simulink model "day06p2"  (R2026a)
settings: Solver=VariableStepAuto  StopTime=inf
InitFcn:
  | input = [9 0 0 0 1 1 0 7 1 0 0 0 4 5 0 3 6 0 2 3 8 4 0 9 9 4 0 6 5 7 0 0 7 7 2 0 8 2 6 0 4 5 2 5 0 1 3 9 1 0 0 9 3 0 1 6 0 0 0 7 0 3 3 0 1 6 9 0 8 3 1 1 0 8 8 0 7 1 0 1 0 0 5 8 0 0 8 0 5 4 0 8 3 0 0 0 7 0 5 4 9 0 0 9 0 6 8 4 0 2 7 0 7 9 1 0 1 2 8 0 2 1 5 0 0 9 8 1 0 4 6 9 0 7 2 0 4 6 0 1 3 9 0 3 0 0 0 9 4 0 0 0 5 3 0 7 6 6 4 0 3 4 0 4 5 0 9 3 0 9 9 0 0 0 9 0 1 5 2 0 5 1 0 8 4 0 1 3 0 4 4 4 8 0 0 0 3 9 0 8 3 0 0 8 2 6 0 8 4 0 4 1 7 0 1 2 6 2 0 4 2 4 5 0 5 2 3 0 0 6 0 3 9 9 0 0 8 3 0 0 2 0 2 8 5 0 7 9 0 0 3 8 0 0 0 9 1 0 6 0 0 2 7 8 0 5 0 0 7 4 0 5 0 0 0 0 2 0 7 8 5 6 0 4 3 0 1 5 6 0 9 0 0 0 9 8 0 9 5 4 4 0 3 4 5 0 1 9 8 0 6 6 0 1 0 0 5 8 0 3 9 0 3 0 0 0 0 9 0 4 8 0 3 2 1 0 6 0 0 6 6 5 7 0 8 0 0 6 7 5 0 4 2 6 4 0 5 0 0 0 2 4 2 1 0 0 3 7 0 2 6 8 0 6 0 0 0 7 3 9 0 5 2 8 0 9 5 0 0 3 4 4 0 4 3 9 0 9 1 0 9 7 4 0 0 4 6 0 0 3 5 0 9 9 0 8 9 0 1 7 2 0 7 4 0 6 1 2 0 0 0 8 0 0 8 3 0 9 6 3 0 0 9 0 0 1 8 0 4 9 0 6 6 0 7 2 9 0 1 5 9 0 2 3 6 0 7 2 0 4 2 7 0 8 1 0 5 8 1 0 6 4 0 7 7 0 2 7 7 0 7 7 0 0 0 8 0 3 6 0 4 6 0 6 4 1 0 0 8 0 4 0 0 5 0 0 9 2 4 4 0 0 0 8 0 4 3 0 2 5 0 3 0 0 0 0 7 7 6 4 0 8 3 0 0 1 2 0 7 6 8 0 9 2 0 9 8 0 5 4 0 7 1 0 9 0 0 0 9 8 0 5 7 0 2 7 0 0 4 1 8 0 0 0 1 0 0 0 0 4 0 2 2 0 6 9 2 0 8 9 0 1 0 0 2 1 3 3 0 0 6 3 0 0 0 4 0 2 9 8 6 0 7 8 0 0 0 6 6 0 3 1 4 0 9 1 2 0 0 5 0 9 8 0 0 3 0 7 6 2 0 1 1 7 0 1 0 0 6 4 5 0 6 2 0 2 8 0 3 3 0 9 0 0 0 0 9 3 2 0 1 1 0 1 8 0 7 0 0 0 7 2 0 9 7 9 0 6 9 3 0 2 2 7 4 0 0 9 0 7 4 8 8 0 8 5 6 0 4 7 2 1 0 5 9 7 1 0 5 9 1 0 0 1 0 7 2 0 2 0 0 0 1 3 1 0 0 0 0 7 0 4 4 0 0 1 3 0 2 6 0 6 9 0 8 7 0 5 0 0 5 6 6 7 0 7 8 4 0 0 0 0 8 0 0 8 1 0 0 2 7 0 2 8 0 0 0 9 3 0 8 8 0 0 0 7 0 6 2 0 3 9 9 0 8 5 1 0 0 9 6 3 0 5 2 0 7 9 2 0 0 2 1 0 1 0 0 0 1 7 0 0 6 7 0 1 9 3 0 1 8 9 8 0 9 6 0 5 9 0 0 4 3 0 0 0 2 4 0 8 5 0 0 1 5 0 0 4 0 8 3 2 0 3 2 0 0 0 2 0 4 3 9 0 0 0 2 5 0 0 2 0 0 7 0 9 7 0 0 0 3 0 0 4 0 8 1 9 0 7 0 0 0 6 3 0 8 4 3 1 0 0 0 7 8 0 0 0 2 0 1 2 3 9 0 9 6 2 0 4 3 0 1 3 0 0 0 0 0 9 1 0 2 1 0 8 5 9 3 0 6 3 0 2 0 0 0 3 0 0 5 0 1 4 0 0 2 6 7 0 7 9 1 1 0 1 7 2 0 3 6 7 9 0 0 0 7 0 4 3 0 9 9 4 0 4 0 0 0 0 3 4 0 2 7 4 0 3 5 0 6 0 0 0 3 3 8 8 0 0 0 6 0 0 2 6 0 1 9 9 0 8 1 0 9 9 0 0 4 0 0 8 6 0 8 7 0 1 6 2 0 0 4 2 0 9 0 0 9 8 0 0 9 2 0 5 3 1 0 7 8 6 0 5 2 0 0 1 9 0 8 9 0 1 3 0 0 0 8 1 6 7 0 0 1 0 7 4 0 4 7 5 0 6 1 0 0 0 7 0 3 6 7 2 0 8 6 0 5 5 0 9 6 0 1 2 0 7 9 7 3 0 1 5 9 0 0 1 0 8 9 0 6 3 9 0 1 9 6 0 3 9 0 6 8 0 6 8 4 0 0 2 5 0 3 0 0 0 7 4 0 8 0 0 9 0 0 0 7 0 0 2 3 7 0 3 7 0 3 2 0 1 0 0 0 0 4 9 1 0 0 9 6 0 2 7 2 0 0 8 0 2 7 7 0 1 3 4 0 0 3 0 0 7 0 6 2 4 0 3 4 9 7 0 2 2 2 0 4 4 0 7 0 0 2 0 0 0 0 0 4 4 0 5 9 0 5 6 4 6 0 2 2 7 0 3 6 6 0 3 4 9 0 1 0 0 9 8 0 8 0 0 0 5 0 0 0 3 6 0 4 1 0 5 4 0 0 9 8 0 0 3 0 1 8 7 0 4 4 6 0 0 5 0 4 2 2 0 4 6 0 0 3 5 0 6 8 8 0 1 0 0 0 4 6 2 0 0 0 3 0 8 5 4 0 3 1 0 9 2 5 8 0 4 6 0 0 0 0 3 5 0 3 3 0 0 5 7 0 5 3 6 0 2 9 9 0 9 3 0 8 5 4 6 0 7 8 6 0 8 5 2 1 0 8 7 0 4 7 0 3 1 0 0 0 2 0 0 4 0 7 2 0 0 1 0 0 3 6 0 5 3 6 0 2 0 0 6 5 9 0 8 6 0 0 0 4 1 1 0 6 6 0 6 0 0 6 0 0 7 9 7 7 0 0 5 0 4 1 0 9 5 5 0 8 0 0 3 2 0 0 9 9 5 0 5 7 0 0 9 5 0 2 8 5 4 0 8 2 0 0 9 6 4 0 2 1 3 0 1 1 0 4 4 0 8 1 6 4 0 6 1 0 0 0 9 3 3 0 6 7 0 5 1 0 1 2 7 0 1 0 0 0 0 0 4 0 5 0 0 4 2 0 5 7 0 3 3 8 3 0 0 9 0 0 0 7 0 7 5 4 0 9 1 6 0 3 7 0 1 8 8 0 2 8 0 0 6 8 1 4 0 9 0 0 5 5 0 0 0 5 7 0 9 6 0 0 2 4 0 1 0 0 0 0 6 0 2 3 3 0 5 6 0 3 7 0 4 9 0 7 8 0 6 4 0 5 3 7 0 2 7 7 0 0 4 0 0 0 4 8 0 2 5 3 7 0 0 5 4 0 0 0 3 0 2 2 1 0 1 6 0 3 4 0 8 6 4 0 4 1 0 0 0 0 6 0 8 6 1 7 0 8 1 6 0 1 1 0 0 9 0 0 3 4 0 7 0 0 4 3 1 3 0 4 5 0 4 6 7 0 1 5 0 8 4 8 8 0 0 0 2 0 7 9 0 2 2 6 0 0 7 0 6 0 0 0 6 6 0 0 7 5 9 0 0 0 8 0 2 5 7 0 1 6 4 0 7 9 0 2 8 8 0 0 1 3 6 0 0 8 1 0 4 9 7 7 0 4 8 2 0 0 8 0 0 7 0 7 9 0 1 4 2 0 1 8 0 7 6 0 4 1 0 4 4 5 7 0 6 3 0 5 5 1 5 0 3 4 0 7 9 0 0 0 1 0 3 5 0 0 5 8 3 0 0 4 1 0 1 7 9 8 0 5 8 3 0 6 7 0 5 8 1 0 1 5 0 0 7 0 5 4 0 5 1 0 9 6 0 0 5 2 0 2 2 5 0 4 9 5 0 0 0 8 0 6 7 0 4 0 0 0 8 1 9 9 0 8 4 1 0 9 2 5 4 0 2 7 1 0 9 4 2 0 3 8 7 0 4 5 2 0 8 2 4 0 5 3 8 0 1 4 0 9 6 9 0 4 2 0 4 6 5 0 2 2 0 2 1 0 8 3 8 9 0 5 4 8 0 0 8 8 0 2 5 0 8 7 8 0 5 7 9 0 2 7 3 6 0 9 0 0 0 0 1 0 4 2 0 5 3 3 0 7 8 7 0 8 5 8 0 4 0 0 0 5 3 0 3 5 2 0 0 6 0 5 2 0 6 7 9 0 0 2 0 0 0 7 4 3 0 1 3 6 0 5 3 0 2 6 0 9 6 0 7 5 3 0 7 3 0 7 2 0 1 9 0 9 1 0 2 5 7 0 1 9 0 2 3 4 0 4 6 0 8 1 0 0 2 7 1 3 0 5 8 5 0 4 7 7 0 3 2 4 0 0 4 8 0 1 7 5 7 0 0 0 5 1 0 0 0 0 5 0 1 5 0 8 0 0 3 1 4 0 3 2 0 0 8 4 0 3 0 0 4 5 4 0 6 8 3 0 0 7 0 6 5 0 6 2 0 4 1 0 2 6 8 7 0 5 1 4 0 4 2 3 0 6 2 0 3 4 4 0 5 0 0 8 1 0 5 1 0 7 9 7 0 0 3 3 7 0 7 6 6 7 0 7 2 2 0 7 2 7 0 0 1 0 7 6 0 5 9 2 0 7 7 0 1 3 0 3 7 6 0 0 4 8 0 9 4 0 4 8 0 3 0 0 9 0 0 0 0 0 7 0 8 8 0 3 6 0 8 1 3 0 3 7 3 0 6 6 5 0 9 4 7 8 0 9 8 4 0 2 3 0 0 0 0 4 0 0 0 4 0 2 5 8 5 0 5 3 0 8 8 9 0 0 3 0 6 9 0 0 0 5 6 0 6 2 0 1 3 0 1 8 4 0 4 3 0 8 0 0 0 0 0 0 9 0 0 7 0 4 5 8 0 5 0 0 0 2 8 4 0 6 2 0 6 9 3 1 0 4 8 0 7 0 0 9 6 3 0 1 0 0 0 3 0 0 3 6 0 0 7 1 0 1 9 9 3 0 7 9 5 0 7 0 0 0 9 4 5 0 0 8 8 0 0 0 0 8 0 1 5 1 9 0 6 2 4 0 0 3 8 0 7 6 2 0 1 4 0 0 0 2 0 1 4 3 0 6 2 0 0 7 4 0 1 8 0 0 0 7 0 8 2 0 3 6 0 1 9 2 0 8 8 5 0 4 8 1 0 5 7 8 0 7 8 7 0 2 4 1 2 0 2 9 0 0 9 4 0 7 2 7 0 9 1 9 0 2 6 0 0 0 1 3 0 8 5 4 0 7 5 4 0 5 2 2 0 2 3 0 0 4 5 0 9 0 0 0 2 9 8 0 1 3 0 0 0 0 8 1 0 5 6 0 4 9 3 0 6 7 0 6 3 6 0 1 3 1 0 1 6 5 0 0 2 3 0 0 5 0 9 1 2 0 2 4 0 2 2 3 0 6 5 5 0 0 5 0 0 6 8 0 0 3 0 4 9 5 0 1 9 4 0 0 9 4 5 0 3 7 1 0 8 0 0 3 5 0 0 0 1 3 0 0 7 7 0 1 9 0 6 8 2 7 0 6 1 4 0 6 4 6 0 8 1 6 0 0 1 0 0 0 0 9 0 4 6 6 0 2 5 7 0 9 1 0 0 6 2 0 0 3 7 0 0 5 0 9 7 7 0 2 4 7 4 0 9 8 0 8 4 2 0 0 8 4 0 8 1 1 0 0 9 0 1 2 0 8 1 5 0 0 2 0 8 1 0 7 1 0 0 4 2 0 0 3 1 0 6 9 2 0 5 1 7 0 8 7 2 0 8 8 2 0 0 0 0 7 0 6 4 0 1 7 1 4 0 2 7 0 6 9 0 0 8 0 4 1 0 8 2 8 3 0 1 5 0 1 4 0 6 2 0 8 5 0 0 7 3 0 0 0 9 1 0 7 7 0 7 9 0 2 7 5 0 0 6 4 0 0 8 7 5 7 0 2 4 7 0 6 9 1 1 0 5 4 0 5 4 4 0 6 7 0 0 6 3 0 4 6 1 4 0 0 0 0 2 0 2 5 2 0 2 4 6 0 3 1 5 0 8 0 0 0 0 5 1 0 7 9 4 0 3 5 0 5 1 0 2 8 0 3 6 6 0 5 4 0 6 9 0 4 1 0 3 4 9 0 5 7 0 9 9 3 0 9 0 0 7 4 0 8 1 0 4 2 0 4 4 0 4 0 0 5 6 0 0 0 1 0 8 8 0 9 1 0 0 5 8 3 0 0 0 8 0 6 6 0 9 7 9 0 9 1 3 0 0 2 0 6 2 7 0 4 2 0 9 9 9 6 0 9 4 9 0 0 0 9 0 7 1 0 0 0 3 1 0 0 1 3 0 2 7 0 9 6 6 3 0 9 3 6 0 3 5 0 0 9 5 3 0 5 4 0 3 3 0 0 5 2 0 0 0 3 8 0 7 7 0 3 7 7 0 8 0 0 9 1 0 0 1 0 7 5 0 8 9 4 0 9 7 7 4 0 0 3 2 0 0 9 3 0 5 1 0 9 4 0 9 4 3 0 7 5 6 0 3 0 0 8 4 0 0 0 9 0 2 1 0 0 0 9 8 0 9 8 2 0 9 3 9 0 5 1 0 6 7 0 5 4 0 4 3 0 0 1 3 9 0 5 3 0 0 7 3 4 0 0 7 0 4 9 0 2 9 3 5 0 0 7 0 0 8 0 0 0 6 8 0 0 7 8 0 6 7 0 0 1 0 3 0 0 0 0 9 0 8 0 0 6 6 5 0 8 6 0 7 7 4 5 0 4 4 5 7 0 2 4 0 3 9 0 3 9 1 0 2 7 0 8 8 0 0 5 0 0 0 5 3 0 3 1 0 4 4 0 0 7 0 9 6 0 0 7 5 0 3 3 4 1 0 9 2 9 0 0 0 5 7 0 4 5 0 2 5 0 7 2 0 0 0 0 6 0 9 9 0 0 6 5 0 9 9 0 3 5 9 0 0 7 5 0 8 2 7 0 1 5 0 3 5 1 0 0 6 9 0 4 1 0 3 0 0 0 8 0 6 0 0 8 6 2 0 4 6 0 9 8 3 8 0 2 8 0 4 4 0 4 7 0 2 6 3 0 2 8 0 4 0 0 0 0 7 8 0 0 4 0 5 6 0 0 2 2 3 0 0 1 0 0 8 0 0 8 1 0 6 1 0 3 0 0 4 1 6 0 4 1 9 0 8 4 7 6 0 2 1 0 7 1 4 0 1 5 8 0 8 2 0 0 8 0 0 1 0 0 0 7 0 0 2 2 8 0 9 1 1 0 4 6 6 3 0 6 6 1 0 1 5 0 1 2 6 1 0 0 0 6 3 0 0 0 8 0 3 4 9 0 2 6 0 9 5 0 9 3 0 9 1 9 4 0 5 9 0 2 2 4 0 1 6 8 9 0 3 3 0 7 8 0 6 3 0 3 6 1 0 4 1 4 0 0 2 3 0 8 6 0 9 0 0 0 0 4 0 8 6 4 0 7 3 2 0 4 9 0 1 3 3 0 4 4 9 0 0 4 0 0 7 2 0 0 3 0 9 7 0 0 0 8 3 0 0 9 0 5 4 0 0 6 3 0 6 0 0 0 0 7 0 8 1 7 1 0 9 8 6 4 0 8 8 4 0 4 4 8 0 8 7 1 0 8 6 5 0 9 4 0 0 0 7 2 0 5 7 6 0 9 9 0 5 2 0 0 3 0 0 5 8 0 0 0 7 2 0 8 9 4 0 1 5 0 6 6 0 7 2 0 5 5 2 7 0 6 0 0 0 9 4 0 0 1 0 0 5 5 9 0 0 0 5 0 1 7 5 0 8 5 0 3 9 0 0 0 3 0 2 7 0 0 5 0 7 0 0 9 2 0 0 0 0 8 0 7 2 8 0 0 0 3 0 8 0 0 0 4 7 3 0 2 7 4 0 0 3 4 0 7 2 0 5 6 9 9 0 3 9 0 9 2 0 5 4 4 7 0;
  |     1 5 0 0 9 5 0 6 8 6 0 0 6 3 0 6 5 0 2 7 9 7 0 7 8 5 0 7 7 2 8 0 2 4 4 0 7 7 6 0 1 8 7 9 0 2 5 7 0 0 0 9 7 0 7 1 0 0 8 7 0 2 7 0 4 5 0 0 3 3 8 3 0 2 5 0 8 6 0 1 6 0 2 5 0 6 6 0 1 5 0 1 8 0 5 8 4 0 5 7 1 0 3 5 0 9 3 2 0 4 8 0 9 6 7 0 6 2 6 0 9 3 9 0 0 8 4 2 0 7 9 5 0 1 6 0 1 3 0 4 5 4 0 5 3 0 4 3 3 0 0 2 6 3 0 8 4 5 8 0 9 2 0 6 1 0 4 1 0 1 4 5 0 0 5 0 6 4 9 0 7 9 0 8 4 0 2 0 0 3 5 1 5 0 0 7 6 4 0 6 9 0 0 8 7 6 0 4 8 0 6 5 3 0 8 8 9 9 0 4 3 1 3 0 9 3 0 0 3 1 0 8 2 8 0 0 9 1 0 9 3 0 4 6 8 0 8 4 0 1 7 7 0 0 9 2 8 0 9 5 0 0 7 7 0 7 8 0 4 9 0 8 7 0 0 0 7 0 5 4 9 9 0 6 6 0 7 8 5 0 3 9 0 0 3 2 0 5 2 2 6 0 5 5 0 0 0 2 8 0 2 5 0 9 4 0 8 8 0 4 1 0 2 6 2 0 6 6 0 6 1 0 8 8 6 0 1 4 0 0 1 3 7 0 5 2 0 8 7 4 0 7 1 7 9 0 8 2 1 0 6 5 5 6 0 0 6 7 0 7 9 9 0 8 8 0 0 9 8 6 0 8 5 6 0 7 4 4 0 7 3 3 0 5 2 7 0 8 7 0 6 2 4 7 0 7 6 8 0 4 6 0 5 1 0 1 9 0 1 5 3 0 9 7 0 6 1 1 0 0 0 3 0 3 5 3 0 7 9 8 0 0 9 0 7 4 9 0 2 8 0 4 1 0 0 4 8 0 1 5 5 0 6 9 1 0 1 2 0 3 3 4 0 4 1 0 6 1 4 0 3 7 0 2 2 0 1 7 2 0 3 4 0 1 6 4 0 3 7 0 8 4 0 6 2 6 0 8 6 0 4 6 0 7 0 0 5 5 4 9 0 5 4 8 0 6 8 0 0 3 0 3 5 0 0 0 7 6 6 8 0 9 9 0 0 8 7 0 9 7 8 0 0 7 0 1 4 0 5 6 0 1 3 0 6 7 9 0 0 1 0 7 2 0 3 2 3 0 9 8 8 0 0 9 6 0 8 8 3 6 0 9 6 0 6 9 7 0 4 0 0 2 3 0 6 2 5 4 0 0 5 4 0 0 3 7 0 9 8 9 1 0 5 2 2 9 0 4 4 0 4 8 4 0 5 9 8 0 2 6 0 1 9 0 0 3 0 5 5 0 0 3 7 8 0 9 0 0 6 1 0 0 3 9 0 8 3 0 1 5 0 3 7 1 8 0 5 3 6 0 4 6 0 9 3 0 9 3 0 0 6 6 0 3 9 6 0 4 8 5 0 2 3 3 7 0 0 6 0 2 3 5 6 0 1 1 2 0 2 8 5 2 0 4 2 9 2 0 2 2 6 0 5 3 0 7 4 0 7 1 0 0 5 1 6 0 0 0 6 7 0 1 7 0 0 4 0 0 9 2 0 4 1 0 7 5 0 5 0 0 1 5 3 8 0 6 1 6 0 0 0 0 2 0 9 7 6 0 2 1 6 0 1 5 0 6 8 7 5 0 8 6 0 0 2 2 0 8 2 0 9 6 7 0 9 4 1 0 0 5 8 0 0 7 7 0 4 6 4 0 0 4 6 0 2 5 0 0 5 7 2 0 6 8 0 7 6 5 0 1 7 5 6 0 7 9 0 2 6 7 0 2 7 2 0 0 5 8 0 8 1 9 0 2 9 0 0 6 0 1 7 6 0 5 1 0 0 0 3 0 7 6 4 0 7 9 1 1 0 8 2 0 0 5 0 4 4 0 0 5 5 0 0 8 0 2 8 5 0 7 6 8 0 9 1 0 6 6 4 0 0 0 8 9 5 0 4 5 4 0 7 4 2 1 0 9 2 2 0 5 5 0 2 8 2 1 0 0 8 1 6 0 2 7 0 5 9 6 0 0 9 7 0 5 0 0 5 4 0 0 7 0 8 7 0 0 9 4 7 0 7 4 9 0 0 1 3 8 0 4 8 2 6 0 0 0 9 0 2 7 0 1 5 9 0 7 1 5 0 0 4 4 0 0 5 2 0 4 7 0 5 4 0 0 0 1 1 7 0 6 1 2 0 8 8 3 0 3 9 3 0 5 6 0 6 2 0 0 1 5 0 2 1 0 4 7 0 0 6 1 0 0 2 4 0 7 6 0 3 7 0 0 9 9 0 9 7 9 0 1 2 9 0 5 5 0 6 1 1 0 6 9 0 5 9 1 0 0 8 6 7 2 0 0 2 0 6 3 0 7 2 1 0 2 2 0 0 0 9 0 8 8 8 6 0 6 7 0 6 8 0 6 2 0 7 5 0 6 5 3 8 0 5 8 4 0 0 2 0 5 7 0 4 9 4 0 2 6 2 0 8 3 0 9 4 0 3 5 5 8 0 8 9 0 8 1 9 0 7 3 0 5 0 0 1 3 0 7 8 0 0 1 2 5 0 3 6 0 8 7 0 5 8 5 0 0 2 8 2 0 0 5 3 0 7 7 8 0 1 6 0 6 8 5 0 1 7 9 0 0 9 0 0 9 0 5 1 8 0 2 1 5 2 0 8 4 1 0 4 3 0 1 3 0 7 7 0 0 0 0 7 1 0 4 1 0 2 1 5 3 0 6 1 3 0 5 8 1 0 3 3 2 0 8 1 0 7 6 0 7 0 0 0 3 2 0 2 8 7 0 7 1 0 6 2 9 0 6 4 0 0 6 0 9 8 6 0 4 4 6 0 0 8 0 4 5 8 0 3 1 0 0 4 7 0 2 5 8 0 1 6 1 0 0 2 8 0 8 5 6 0 2 4 2 0 3 9 0 2 3 3 8 0 3 1 0 0 6 9 7 6 0 8 3 6 0 9 0 0 5 1 6 0 7 1 3 0 1 9 0 3 4 3 1 0 2 6 3 0 4 7 2 0 0 3 4 0 3 5 0 7 8 0 0 4 1 0 5 5 0 4 7 0 0 9 1 0 5 9 0 5 8 5 0 5 9 0 4 6 7 0 2 4 8 0 0 4 5 4 0 2 8 0 4 0 0 9 0 0 5 4 1 5 0 5 5 0 6 5 0 9 9 8 0 9 2 0 3 9 0 0 4 7 7 0 9 7 0 8 6 8 0 9 2 6 2 0 0 4 0 8 1 9 2 0 1 6 7 0 4 9 0 2 6 0 4 1 2 0 0 1 1 7 0 0 5 7 6 0 2 1 0 3 1 0 4 3 8 0 4 0 0 0 0 0 8 0 4 0 0 2 7 0 8 7 0 5 4 2 1 0 0 6 0 0 9 3 0 3 4 1 0 5 2 5 0 1 8 0 7 6 0 0 6 6 8 0 6 9 3 3 0 3 8 0 1 1 0 2 4 5 5 0 8 5 0 0 2 6 0 2 0 0 0 5 7 0 8 9 2 0 3 6 0 4 8 0 5 0 0 7 8 0 3 8 0 8 7 3 0 8 7 5 0 9 9 0 5 3 7 3 0 5 6 4 8 0 6 2 2 0 8 6 3 0 1 4 9 0 1 5 0 0 3 0 9 4 1 0 4 5 0 0 0 7 8 0 1 3 8 4 0 6 7 4 0 8 9 0 7 9 0 0 6 4 0 2 0 0 6 9 9 5 0 7 5 0 3 6 8 0 3 3 0 6 5 5 5 0 3 9 9 0 6 7 0 5 3 0 0 0 3 0 9 4 0 0 2 3 0 0 9 7 8 0 0 6 2 0 5 1 1 0 2 7 1 0 4 4 0 6 2 7 0 3 5 5 3 0 0 8 1 0 9 8 7 8 0 8 6 5 0 2 6 0 7 8 0 4 3 0 5 9 3 0 8 7 0 2 2 0 2 3 0 1 3 3 8 0 5 7 0 0 4 1 1 0 1 8 0 3 4 1 0 0 1 0 8 6 6 0 9 5 1 0 1 7 1 0 2 1 7 1 0 2 9 5 0 3 8 0 2 4 6 0 4 1 0 8 7 0 2 7 0 6 9 0 3 3 0 0 6 1 0 5 7 4 0 8 5 6 3 0 0 5 0 8 9 0 2 3 7 0 8 1 2 3 0 7 9 2 0 1 2 1 3 0 8 3 7 0 1 1 3 0 8 7 6 0 9 5 8 0 3 3 7 0 9 1 9 0 2 4 0 4 2 2 0 2 4 0 4 4 1 0 8 9 0 3 4 0 1 3 3 1 0 2 7 4 6 0 9 8 0 4 3 0 5 2 8 0 8 5 8 0 8 7 5 8 0 3 1 0 0 0 4 0 9 8 0 5 7 6 0 0 3 3 0 5 9 3 0 4 0 0 0 5 6 0 8 2 5 0 5 6 0 3 8 0 6 6 9 0 0 6 3 5 0 4 2 1 0 9 4 1 0 4 5 0 4 4 0 8 5 0 7 6 8 0 4 4 0 6 5 0 6 3 0 5 6 0 7 1 1 0 7 5 0 6 2 0 0 4 5 0 8 7 2 0 7 8 4 2 0 9 5 2 0 9 2 6 0 2 3 6 0 3 7 8 0 2 7 6 1 0 0 9 2 7 0 0 3 6 1 0 5 2 0 7 0 0 4 2 3 0 7 2 0 3 4 7 0 9 0 0 1 7 7 0 5 8 9 0 5 2 0 3 9 0 2 8 0 4 1 0 4 1 5 0 0 8 1 3 0 1 3 8 0 9 5 0 3 3 0 0 6 0 0 8 8 0 0 3 0 9 3 7 0 6 8 6 4 0 9 5 8 4 0 9 5 9 0 5 3 2 0 7 4 0 3 3 0 4 2 1 0 4 5 0 4 9 0 7 4 2 0 0 3 9 0 8 8 0 1 8 0 8 0 0 8 5 0 0 0 9 1 0 5 1 0 3 8 0 3 9 6 0 1 4 3 0 6 5 4 0 5 9 2 3 0 6 1 5 0 6 3 0 0 0 0 7 0 0 5 9 0 3 6 9 2 0 1 6 0 7 8 5 0 8 2 0 1 9 0 0 0 6 3 0 5 5 0 4 8 0 1 8 2 0 4 3 0 3 7 8 0 9 1 5 6 0 5 3 0 0 5 9 0 7 2 0 0 1 9 0 0 5 3 0 2 2 7 9 0 3 2 0 2 0 0 8 7 6 0 1 0 0 0 5 0 0 1 1 0 0 7 9 0 5 8 1 6 0 5 5 8 0 5 3 6 0 3 6 4 0 2 7 8 0 0 0 2 8 0 9 4 4 4 0 9 4 8 0 0 7 5 0 6 7 3 0 7 2 0 0 8 9 0 5 7 8 0 8 4 1 0 8 4 0 9 7 4 0 0 2 0 9 3 0 7 5 0 7 4 4 0 3 4 5 0 5 7 5 0 0 1 4 0 9 7 7 0 9 4 6 8 0 1 1 0 0 7 7 0 6 7 3 0 9 1 2 0 7 0 0 0 0 5 6 0 8 8 1 0 2 4 4 0 9 7 7 0 7 7 2 0 3 7 0 5 1 2 0 2 9 1 0 4 6 2 0 0 0 1 8 0 5 9 0 3 1 7 0 5 4 0 5 5 4 0 2 6 7 0 4 2 9 0 0 9 6 0 0 5 0 1 9 2 0 6 3 0 1 2 8 0 9 8 1 0 0 5 0 9 8 2 0 0 1 0 1 8 5 0 4 8 9 0 0 4 8 8 0 0 9 3 0 4 3 0 2 6 3 0 0 1 4 3 0 9 6 0 1 8 0 7 1 6 4 0 0 8 6 0 2 5 7 0 1 8 3 0 0 5 0 0 1 2 5 0 1 2 9 0 3 3 3 0 2 8 0 0 8 7 0 3 3 7 0 0 2 0 6 4 6 0 8 9 9 4 0 2 4 0 2 9 0 0 7 9 8 0 0 7 9 0 0 5 0 0 9 0 4 8 4 0 7 6 0 5 8 0 1 7 0 0 1 5 0 0 1 1 0 8 6 5 0 2 7 5 0 2 3 6 0 6 2 7 0 0 0 0 5 0 7 2 0 9 5 9 9 0 7 9 0 8 3 0 0 7 0 4 9 0 2 3 2 8 0 9 6 0 1 8 0 7 7 0 5 6 0 8 9 3 0 0 5 6 1 0 1 2 0 2 1 0 8 3 3 0 0 2 8 7 0 9 2 7 8 0 5 4 6 0 9 3 9 9 0 2 8 0 1 8 4 0 2 9 9 0 3 6 0 9 4 2 6 0 0 7 9 2 0 8 7 6 0 1 6 1 0 4 9 9 0 5 2 0 6 9 9 2 0 8 9 8 0 2 8 0 7 7 0 4 8 0 8 7 4 0 3 3 0 2 3 0 3 3 0 2 5 9 0 8 8 0 6 4 5 0 9 8 0 9 8 0 9 2 0 4 9 0 1 3 0 1 0 0 1 9 0 0 0 3 0 3 9 0 4 5 0 6 2 3 2 0 0 4 3 0 2 4 0 6 3 3 0 7 1 1 0 0 2 0 7 4 4 0 5 1 0 7 6 8 7 0 7 6 6 0 2 4 9 0 6 6 0 7 8 7 8 0 0 1 6 0 4 9 0 9 3 8 9 0 6 6 0 0 6 8 0 0 7 4 5 0 1 2 0 6 6 2 0 5 6 0 3 9 7 1 0 5 4 0 1 4 1 0 4 0 0 1 5 0 0 4 0 9 7 0 7 3 3 0 7 4 5 2 0 5 3 9 0 0 9 1 0 3 8 0 4 3 0 5 7 0 0 2 2 2 0 6 6 0 1 8 0 0 9 8 0 4 2 0 0 1 9 8 0 0 2 7 0 0 3 9 0 6 9 0 5 8 0 1 3 0 1 6 0 7 1 8 6 0 8 8 0 0 3 2 4 0 4 6 0 0 2 0 3 3 8 4 0 0 1 0 7 8 0 0 3 6 7 0 8 5 8 0 7 6 0 0 2 0 4 0 0 0 6 1 0 3 6 0 5 3 7 0 9 1 0 6 2 6 6 0 8 2 3 5 0 8 7 0 3 4 0 8 1 8 0 9 9 0 2 1 0 3 1 0 0 0 5 3 0 1 1 0 4 1 0 5 4 0 3 4 5 0 5 7 0 7 1 1 0 0 3 2 0 0 4 1 1 2 0 8 4 0 4 5 0 2 3 0 0 0 0 4 0 4 4 3 0 1 8 0 8 8 0 6 9 5 0 3 1 2 0 9 5 8 0 4 6 0 2 7 5 0 5 9 1 0 1 0 0 1 2 0 9 6 0 7 1 0 9 4 1 0 6 7 0 4 8 1 1 0 4 3 0 1 3 0 7 7 0 9 2 3 0 7 3 0 6 7 0 0 0 6 5 0 0 5 0 8 5 6 0 5 9 2 0 1 4 0 7 9 0 0 7 5 0 7 4 0 4 0 0 1 9 7 0 8 3 2 0 9 9 1 2 0 7 3 0 9 2 2 0 9 6 9 0 1 4 3 0 7 0 0 1 8 0 1 6 0 2 8 1 3 0 7 2 8 0 2 9 1 7 0 9 9 6 0 8 3 0 8 3 9 1 0 8 3 6 5 0 0 8 8 0 9 4 1 0 1 2 0 4 5 0 1 9 0 7 8 7 4 0 3 4 0 7 4 5 0 0 7 4 8 0 5 5 0 4 3 0 4 4 0 4 9 9 0 3 1 1 0 1 4 5 0 9 5 0 2 1 0 0 9 6 0 0 9 2 0 9 1 4 0 8 1 0 8 7 9 0 5 4 9 0 5 6 0 8 3 6 0 0 8 0 6 3 0 8 7 8 8 0 7 2 0 3 9 2 0 3 6 0 8 0 0 0 0 2 0 9 5 7 8 0 8 4 3 4 0 9 4 4 0 6 6 4 0 6 7 2 0 9 7 3 0 2 6 0 9 6 3 9 0 4 6 7 0 3 5 0 9 4 4 0 8 8 0 5 9 0 0 0 6 9 0 9 2 6 0 5 6 0 7 8 0 1 2 0 7 4 9 0 0 9 1 0 0 9 9 0 0 6 0 0 9 9 7 0 0 5 2 0 2 1 2 0 4 3 0 5 2 8 0 8 8 0 6 5 0 8 8 0 3 9 0 3 8 8 0 0 0 6 0 9 2 6 0 0 4 2 0 6 7 3 0 1 7 1 0 5 8 6 0 2 2 6 0 5 1 0 7 8 9 9 0 8 3 0 1 4 0 1 6 1 7 0;
  |     8 4 0 0 7 5 0 6 1 9 0 0 7 3 0 9 5 0 0 7 2 2 0 0 6 3 0 7 3 8 1 0 2 7 5 0 0 4 8 0 6 5 2 6 0 1 8 4 0 0 1 6 3 0 8 7 0 4 9 5 0 7 5 0 3 9 0 0 7 7 9 5 0 7 6 0 8 7 0 1 6 0 0 5 0 3 6 0 3 6 0 5 1 0 6 9 6 0 7 2 4 0 8 8 0 0 0 7 0 2 5 0 8 9 5 0 2 7 8 0 7 8 8 0 3 2 5 7 0 8 1 3 0 5 6 0 3 6 0 9 5 0 0 7 1 0 9 5 5 0 7 6 7 5 0 8 9 0 0 0 1 7 0 4 1 0 5 6 0 2 5 4 0 1 8 0 0 4 1 0 2 6 0 8 5 0 1 0 0 6 2 1 4 0 7 5 7 7 0 2 8 8 0 0 9 2 0 1 0 0 6 3 5 0 0 6 5 1 0 2 9 2 5 0 2 7 0 0 7 2 0 8 4 9 0 9 4 3 0 7 3 0 2 3 0 0 7 5 0 2 3 2 0 0 7 8 6 0 6 6 0 0 8 8 0 3 3 0 9 0 0 9 5 0 0 4 3 0 8 8 8 9 0 8 2 0 1 3 0 0 6 7 9 0 3 6 0 0 0 0 6 0 3 3 0 0 0 4 5 0 6 7 0 2 8 0 3 5 0 5 0 0 8 7 7 0 7 5 0 1 1 0 7 9 6 0 7 8 0 0 0 4 8 0 8 4 0 2 6 0 0 6 3 4 8 0 2 8 4 0 3 6 3 4 0 3 3 8 0 1 4 6 0 6 1 6 0 8 2 8 0 1 6 9 0 4 1 9 0 3 1 0 0 2 1 4 0 9 8 0 2 9 5 9 0 2 2 1 0 5 2 0 1 1 0 9 5 0 7 7 3 0 4 0 0 6 1 3 0 0 4 1 0 7 2 8 0 3 4 5 0 5 3 0 4 8 8 0 7 9 0 9 9 0 0 6 9 0 1 4 1 0 7 2 7 0 6 9 0 2 8 2 0 8 4 0 2 9 3 0 7 0 0 0 1 0 9 2 5 0 8 8 0 8 2 7 0 6 6 0 0 9 0 0 6 5 0 3 4 0 1 8 0 4 8 0 6 8 5 5 0 1 2 8 0 3 3 0 0 1 0 9 1 7 0 0 9 6 4 0 0 6 7 0 0 2 6 0 1 6 1 0 0 9 0 8 2 0 3 1 0 2 9 0 6 7 3 0 0 6 0 3 5 0 3 3 1 0 6 3 2 0 6 1 1 0 8 3 5 8 0 9 3 0 4 1 2 0 1 0 0 1 7 0 9 3 3 3 0 0 8 5 0 7 1 6 0 3 9 8 0 0 1 9 4 4 0 9 9 0 8 1 9 0 4 8 1 0 5 8 0 7 7 0 5 9 0 3 9 0 0 3 1 9 0 5 5 0 8 6 0 0 6 6 0 2 6 0 7 5 0 4 9 6 1 0 7 4 5 0 4 3 0 6 2 0 5 6 0 5 6 4 0 3 7 5 0 6 3 8 0 6 9 1 0 0 1 7 0 6 8 2 0 0 1 3 6 0 2 7 6 5 0 5 9 9 4 0 8 4 3 0 1 3 0 4 1 0 5 3 0 0 7 5 5 0 0 3 5 5 0 5 1 6 0 2 0 0 4 8 0 3 5 0 1 2 0 9 2 0 2 9 4 1 0 1 6 6 0 0 2 3 4 0 6 2 6 0 9 7 9 0 2 9 0 4 2 7 3 0 5 5 0 0 5 8 0 0 5 0 4 4 8 0 2 9 4 6 0 9 0 0 0 8 7 0 8 7 4 0 4 3 8 0 4 2 8 0 9 3 2 0 1 4 0 9 2 7 0 4 4 9 4 0 5 8 0 2 1 4 0 7 8 1 1 0 7 9 0 1 3 9 0 0 5 0 2 4 0 3 3 1 0 0 6 0 0 3 1 0 5 8 1 0 7 7 1 3 0 1 3 0 6 7 0 3 7 0 0 6 1 0 6 9 0 6 3 2 0 9 3 1 0 0 7 0 9 2 0 0 0 2 6 6 1 0 5 1 2 0 9 3 1 1 0 4 6 2 0 9 9 0 8 3 7 8 0 8 6 9 7 0 9 1 0 7 1 9 0 0 9 1 0 5 5 0 6 1 0 4 8 0 7 8 1 0 9 6 5 0 7 1 3 0 0 2 7 3 0 2 4 6 9 0 9 2 4 0 9 2 0 5 1 1 0 3 7 1 0 0 7 1 0 0 3 8 0 1 7 0 8 5 2 0 0 0 8 7 0 4 2 5 0 2 3 4 0 7 6 6 0 3 2 0 1 2 0 0 7 2 0 7 7 0 1 6 0 0 4 5 0 0 1 4 0 4 9 0 4 9 1 0 9 1 0 1 9 7 0 2 2 3 0 5 6 0 4 1 9 0 8 8 0 9 9 2 0 0 6 5 1 6 0 1 9 0 0 7 0 0 2 6 0 3 5 0 8 7 1 0 3 2 5 2 0 4 5 0 7 8 0 1 4 0 1 5 0 9 8 7 0 0 0 1 2 0 0 7 0 9 9 0 1 6 5 0 2 7 7 0 9 3 0 5 5 0 3 4 5 7 0 8 9 0 1 7 3 0 3 8 0 3 0 0 2 7 0 9 1 0 0 9 4 5 0 0 1 0 2 1 0 8 2 7 6 0 3 5 2 0 0 4 3 0 4 6 8 0 3 5 0 1 2 0 0 8 9 8 0 3 6 0 3 1 0 2 2 3 0 0 3 3 2 0 5 6 3 0 3 9 0 2 4 0 9 5 0 0 0 6 8 1 0 4 9 0 2 3 8 3 0 2 3 2 0 5 1 4 0 0 7 9 0 2 9 0 4 2 0 4 6 0 0 1 3 0 8 3 8 0 6 4 0 7 3 4 0 7 5 0 4 2 0 9 2 4 0 7 3 0 0 7 7 0 0 8 8 0 4 5 0 0 1 8 0 7 7 0 0 8 4 9 0 0 0 5 0 6 7 7 0 4 7 4 0 3 2 0 4 3 6 7 0 5 4 8 0 8 2 9 2 0 5 9 1 0 2 0 0 6 8 6 0 5 1 8 0 3 5 0 3 5 4 0 0 0 4 9 0 5 5 1 0 0 8 0 0 3 4 0 9 3 4 0 8 9 0 6 3 0 7 1 3 0 7 3 0 9 3 0 1 7 9 0 6 5 0 3 2 1 0 1 3 9 5 0 0 8 3 0 8 7 0 5 0 0 2 0 0 0 2 3 1 0 7 7 0 9 8 0 1 5 3 0 1 8 0 1 7 3 0 6 3 2 0 7 6 0 7 7 1 0 3 7 1 4 0 0 8 0 7 4 7 3 0 3 6 7 0 1 8 0 3 3 0 3 4 6 0 0 3 7 7 0 0 2 1 3 0 4 0 0 9 7 0 9 2 1 0 8 8 2 0 3 6 8 0 3 2 0 7 5 0 2 6 0 0 3 6 4 0 8 9 0 3 4 7 0 4 4 3 0 0 6 6 0 7 8 0 2 9 0 0 3 6 8 0 1 5 2 6 0 5 9 0 6 9 0 5 5 8 3 0 7 8 0 0 8 8 0 8 9 8 0 1 3 0 0 2 5 0 0 8 0 9 2 0 6 0 0 7 7 0 9 8 0 5 5 0 0 1 6 8 0 1 5 0 6 3 1 6 0 4 5 7 8 0 7 7 9 0 3 6 4 0 7 6 0 0 6 6 0 0 7 0 8 5 9 0 5 6 9 0 8 2 8 0 8 2 1 4 0 2 7 9 0 2 4 0 7 7 0 3 2 9 0 5 8 0 0 1 4 6 0 6 1 0 1 8 7 0 5 6 0 0 7 7 9 0 5 9 4 0 6 9 0 1 8 0 0 4 2 0 1 2 1 0 9 7 0 0 1 2 4 0 5 8 1 0 4 7 2 0 3 2 5 0 1 5 0 8 4 8 0 4 2 1 7 0 0 1 6 0 0 3 4 5 0 0 5 1 0 9 3 0 3 2 0 0 3 0 9 7 6 0 1 4 0 2 3 0 7 8 0 3 4 7 4 0 8 9 0 0 0 8 2 0 8 8 0 7 3 9 0 1 9 0 3 6 2 0 9 2 5 0 7 2 5 0 6 4 6 7 0 0 9 2 0 8 3 0 2 8 2 0 1 0 0 9 9 0 8 2 0 6 7 0 3 9 0 6 4 1 0 8 6 0 0 7 7 5 4 0 2 5 0 0 4 0 5 3 5 0 1 5 4 0 0 5 3 2 0 3 9 7 9 0 6 3 7 0 2 7 0 0 5 9 7 0 9 2 0 0 3 9 0 0 8 3 7 0 7 3 0 8 2 8 0 2 9 0 9 5 4 0 5 8 0 9 6 0 1 2 3 0 0 5 5 9 3 0 8 6 0 0 1 0 7 5 7 0 1 1 1 0 3 3 2 4 0 5 2 8 0 2 2 0 8 2 0 7 6 7 0 0 9 2 0 1 4 9 0 8 9 0 1 6 7 0 1 5 2 0 6 7 0 7 9 0 4 7 9 9 0 8 6 5 0 0 7 2 0 0 8 8 0 7 2 0 0 7 0 9 2 0 0 7 8 0 3 5 0 9 4 0 1 4 0 7 8 0 0 0 9 0 6 8 0 1 9 0 0 4 9 0 3 7 8 0 2 9 2 9 0 2 7 7 0 6 9 1 0 2 9 1 0 1 9 2 0 6 4 6 1 0 9 6 8 5 0 7 5 3 7 0 3 3 0 6 5 0 6 1 2 0 3 6 0 9 6 6 0 1 8 0 6 9 3 0 8 4 6 0 2 5 0 8 2 0 6 6 0 6 0 0 6 8 1 0 0 4 4 0 0 2 7 3 0 7 2 0 6 8 0 0 2 3 0 9 5 0 0 7 0 3 8 7 0 4 5 2 1 0 0 0 2 3 0 2 7 1 0 0 5 2 0 7 6 0 2 9 0 2 2 2 0 6 9 0 3 2 0 1 5 8 8 0 1 5 0 1 2 0 5 3 0 2 5 0 8 1 8 0 9 2 1 0 8 4 0 7 1 0 4 9 6 0 4 8 9 0 3 1 1 0 0 3 6 9 0 7 5 3 0 7 6 0 0 0 7 7 0 5 5 3 0 0 6 8 1 0 1 9 0 0 7 3 0 3 6 0 2 6 0 4 5 7 9 0 4 1 0 4 7 0 4 3 8 0 3 3 0 7 1 6 0 6 5 3 5 0 9 7 0 0 2 2 0 7 4 7 0 2 4 0 0 4 4 0 1 5 8 5 0 7 4 0 2 7 0 9 4 8 0 5 6 8 0 2 2 0 1 7 0 0 4 1 0 0 4 4 9 0 5 5 9 0 3 8 9 0 9 4 0 0 7 7 2 0 3 9 6 4 0 0 8 6 9 0 2 7 4 0 0 2 7 0 2 9 3 0 2 2 0 3 9 6 0 1 6 5 0 5 6 7 0 2 4 0 7 8 4 0 6 6 0 1 8 0 4 5 0 4 4 9 0 2 3 2 0 0 7 2 0 0 5 5 0 6 2 9 0 4 6 2 3 0 8 3 0 5 6 6 0 5 3 7 0 9 4 8 0 9 0 0 0 9 3 5 0 1 3 8 0 0 7 5 0 4 2 6 0 6 5 5 0 9 9 0 9 6 9 0 8 4 1 0 2 9 2 0 0 6 7 9 0 3 2 0 9 9 8 0 4 2 0 1 5 3 0 4 1 6 0 8 7 4 0 3 5 1 0 7 6 0 8 3 0 0 3 3 0 0 0 3 0 5 5 7 0 2 8 0 8 7 9 0 3 4 0 0 3 2 0 4 9 6 0 0 5 4 7 0 0 9 8 0 7 8 0 3 4 7 0 0 3 8 7 0 0 2 0 1 4 0 8 7 2 0 0 0 8 4 0 1 7 0 0 5 5 6 0 5 7 0 1 2 5 1 0 7 7 9 0 0 4 3 0 3 9 0 3 5 5 0 6 2 1 0 0 3 0 9 7 8 0 6 9 0 0 0 1 4 0 9 3 0 0 2 4 4 0 0 5 1 0 1 9 0 0 9 0 7 3 8 0 2 4 0 1 6 0 0 9 0 4 5 2 0 2 9 8 0 0 2 7 0 1 8 3 0 2 3 3 0 3 5 2 0 0 0 3 2 0 1 2 0 0 3 2 9 0 9 8 0 6 5 0 8 1 0 9 3 0 6 9 4 5 0 2 8 0 5 8 0 9 6 0 9 8 0 8 6 4 0 0 6 4 8 0 1 7 0 6 8 0 9 8 4 0 0 1 9 1 0 8 4 9 1 0 8 2 6 0 6 5 0 0 0 2 7 0 2 1 2 0 3 3 2 0 8 9 0 0 9 9 4 0 0 8 8 3 0 5 2 1 0 0 1 3 0 2 4 5 0 7 4 0 8 6 8 7 0 5 5 2 0 0 1 0 2 1 0 6 6 0 5 7 8 0 3 2 0 5 9 0 7 5 0 0 7 4 0 0 4 0 9 3 3 0 4 7 0 9 5 0 3 7 0 5 0 0 6 9 0 6 2 0 4 4 4 0 3 8 0 5 1 0 1 1 0 2 5 3 5 0 9 4 8 0 0 2 0 8 7 6 0 7 4 1 0 0 7 0 8 6 4 0 0 4 0 9 8 6 2 0 6 5 9 0 1 6 8 0 8 5 0 5 6 3 7 0 3 9 8 0 6 5 0 0 9 8 7 0 4 5 0 0 1 6 1 0 2 2 1 0 6 4 0 1 6 3 0 3 6 0 3 8 1 4 0 6 3 0 9 6 8 0 1 0 0 7 7 0 4 1 0 1 7 0 9 5 4 0 5 8 6 3 0 2 6 4 0 4 1 4 0 4 6 0 8 6 0 3 5 0 0 6 3 0 0 1 5 0 9 1 0 3 5 8 0 4 3 3 0 4 2 7 0 0 1 5 0 0 8 9 0 8 3 0 0 2 0 3 5 0 6 2 0 9 7 6 4 0 8 7 0 2 4 3 3 0 6 6 0 0 3 0 4 3 1 1 0 9 7 0 4 8 0 8 8 6 6 0 2 8 2 0 6 8 0 2 6 0 6 3 6 0 8 4 0 4 9 0 8 4 1 0 5 9 0 1 1 1 2 0 2 3 6 1 0 9 2 0 7 2 0 9 1 0 0 1 7 0 3 9 0 5 5 0 5 9 6 2 0 4 7 0 9 0 0 3 6 0 1 9 9 0 0 3 0 4 1 1 0 0 5 5 0 0 1 4 7 4 0 6 7 0 4 4 0 5 6 0 1 4 9 6 0 2 6 6 0 4 1 0 2 0 0 0 5 9 0 9 7 3 0 4 5 4 0 2 7 0 0 3 5 0 2 2 8 0 6 0 0 5 9 0 3 1 0 4 5 0 9 7 1 0 5 1 0 0 0 1 9 0 3 9 0 4 0 0 6 1 0 9 3 8 0 6 7 0 5 6 3 0 0 8 4 0 5 3 0 8 9 9 0 2 7 3 0 7 2 0 7 9 0 6 5 2 0 9 5 0 7 5 0 9 6 8 0 3 7 8 0 1 8 3 0 0 8 3 0 7 6 8 0 5 3 0 0 4 8 7 0 3 8 0 4 5 0 9 1 0 3 8 1 1 0 6 6 2 0 2 4 7 0 0 0 9 2 0 3 4 0 0 6 6 1 0 9 9 1 1 0 9 9 8 0 4 3 0 0 7 7 0 6 0 0 2 8 0 5 4 4 1 0 5 6 0 9 2 8 0 0 9 8 1 0 5 1 0 3 8 0 8 3 0 4 2 0 0 4 9 0 0 8 6 3 0 5 4 0 4 4 0 0 4 3 0 0 5 5 0 6 1 4 0 0 8 0 4 9 6 0 9 6 5 0 3 7 0 9 2 3 0 0 4 0 2 3 0 1 7 9 4 0 8 8 0 1 9 4 0 7 5 0 7 8 4 0 1 9 0 0 8 3 6 0 5 9 4 9 0 0 9 5 0 1 5 8 0 6 7 5 0 1 5 2 0 8 8 0 2 8 2 7 0 5 5 5 0 5 1 0 2 8 1 0 8 9 0 7 3 7 0 0 4 2 0 5 5 2 0 0 7 0 4 0 0 6 9 0 5 8 8 0 0 2 5 1 0 3 4 6 0 3 9 0 9 3 6 7 0 7 3 0 0 5 1 0 9 0 0 7 6 4 0 9 9 0 4 1 0 5 3 0 7 9 0 9 2 7 9 0 1 9 0 5 6 9 0 1 9 5 0 8 2 1 0 4 3 0 0 8 8 6 0 8 4 1 0 5 2 0 8 3 4 0 0 5 3 0 3 7 0 1 4 6 5 0;
  |     9 4 2 0 6 0 0 4 3 4 4 0 6 9 0 0 9 0 0 0 3 3 0 0 2 8 0 6 2 4 2 0 3 2 9 0 0 9 9 0 0 1 1 5 0 6 3 0 0 0 7 3 8 0 6 8 0 4 9 8 0 6 4 0 4 6 0 0 6 2 2 6 0 7 9 0 1 7 0 1 8 0 0 4 0 9 5 0 5 5 0 8 8 0 4 8 4 0 0 2 5 0 8 3 0 0 0 4 0 6 3 0 1 3 3 0 1 7 0 0 8 7 8 0 1 5 2 1 0 7 5 8 0 8 3 0 6 0 0 8 4 0 0 6 9 0 8 4 4 0 8 1 6 4 0 7 5 0 0 0 1 5 0 6 9 0 0 2 0 8 2 7 0 7 8 0 0 0 7 0 4 0 0 2 8 0 6 0 0 8 2 1 4 0 5 2 2 1 0 9 2 9 0 0 3 6 0 3 0 0 6 8 2 0 0 9 3 3 0 0 0 4 1 0 5 3 0 0 7 5 0 0 0 2 0 5 6 9 0 7 6 0 3 0 0 0 9 4 0 5 1 5 0 7 5 9 7 0 2 8 0 0 0 6 0 5 7 0 6 0 0 6 4 8 0 6 2 0 2 1 8 0 0 7 9 0 3 7 0 0 1 7 9 0 6 6 0 0 0 0 4 0 2 6 0 0 0 2 4 0 3 8 0 6 8 0 4 4 0 8 0 0 6 2 2 0 4 5 0 4 9 0 6 6 0 0 2 8 0 0 0 0 7 0 8 5 0 7 0 0 0 9 4 1 0 0 8 3 4 0 8 2 2 8 0 1 9 3 0 4 9 4 0 2 4 6 0 4 4 0 0 6 4 5 0 3 8 8 0 6 5 0 0 0 3 6 0 3 0 0 1 6 4 8 0 7 4 4 0 8 3 0 0 5 0 1 8 0 0 0 8 0 7 0 0 1 3 8 0 8 1 5 0 2 2 4 0 1 3 5 0 8 2 0 9 5 5 0 0 3 0 2 9 0 0 2 4 0 0 0 9 0 9 5 5 0 6 5 0 7 3 5 0 5 6 0 7 9 1 0 8 0 0 0 8 0 1 9 6 0 8 1 0 5 5 8 0 8 9 0 0 6 0 0 0 2 0 9 9 0 5 6 0 4 4 0 0 0 4 8 0 9 5 7 0 7 5 0 0 9 0 1 3 9 2 0 6 0 0 0 0 8 4 2 0 7 1 0 1 9 9 0 0 7 0 2 7 0 3 9 0 4 5 0 5 4 5 0 0 8 0 5 5 0 4 9 6 0 0 1 8 0 4 6 3 0 5 6 8 1 0 7 3 0 0 7 9 0 1 0 0 3 1 0 8 7 5 1 0 4 9 5 0 8 5 1 0 2 0 0 0 0 2 2 6 9 0 5 2 0 8 1 9 0 6 9 4 0 3 7 0 4 9 0 2 7 0 9 0 0 0 9 6 5 0 3 9 0 4 0 0 0 3 9 0 3 9 0 7 6 0 7 4 8 4 0 1 9 9 0 3 9 0 0 7 0 8 3 0 7 6 1 0 0 1 6 0 3 0 0 0 7 1 0 0 0 4 4 0 4 9 0 0 0 7 3 0 0 0 0 0 1 0 0 3 9 5 0 8 6 0 0 4 5 0 0 3 0 3 7 4 0 8 5 3 3 0 3 8 8 0 8 2 2 0 7 0 0 4 3 0 9 7 0 6 3 0 4 6 0 9 2 6 8 0 2 5 0 0 4 9 9 2 0 1 2 5 0 8 9 1 0 7 5 0 4 4 2 5 0 0 2 0 2 2 1 0 0 9 0 7 2 1 0 2 2 7 4 0 1 0 0 0 4 7 0 9 2 4 0 8 3 2 0 2 7 2 0 8 4 5 0 3 3 0 9 0 0 0 0 0 0 9 0 7 7 0 2 4 3 0 3 8 2 6 0 0 9 0 1 3 8 0 0 8 0 4 7 0 3 7 0 0 0 3 0 6 2 5 0 9 4 7 0 8 4 5 7 0 8 8 0 5 4 0 6 7 6 0 9 6 0 8 1 0 4 5 7 0 1 4 9 0 0 1 0 8 0 0 0 0 1 5 8 8 0 3 1 8 0 6 6 7 0 0 2 7 3 0 4 4 0 6 2 1 7 0 5 3 6 9 0 0 4 0 3 0 0 0 0 5 6 0 6 2 0 8 1 0 9 7 0 1 3 3 0 9 4 7 0 5 8 2 0 0 0 6 9 0 0 0 0 4 0 8 6 8 0 0 2 0 0 6 3 0 1 2 9 1 0 4 1 0 0 7 2 0 9 4 0 8 3 5 0 0 0 6 8 0 8 1 6 0 7 6 1 0 7 7 4 0 6 8 0 2 5 4 0 7 6 0 6 8 0 1 6 0 0 9 7 0 7 8 9 0 7 7 0 9 8 6 0 7 6 0 4 5 9 0 0 2 4 0 8 6 0 9 7 4 0 3 0 0 6 4 2 9 0 0 7 8 2 0 6 4 0 0 2 0 0 9 1 0 4 4 0 1 3 7 0 7 8 0 0 0 5 7 0 8 6 0 0 4 0 7 3 0 3 3 5 0 0 0 0 8 0 7 5 0 7 4 0 0 5 2 0 0 0 6 0 8 5 0 9 0 0 9 2 3 3 0 1 3 0 3 1 8 0 4 0 0 7 6 0 9 7 0 4 4 0 7 4 9 4 0 0 5 0 6 9 0 9 9 9 1 0 7 8 1 0 3 3 4 0 9 7 2 0 6 7 0 8 0 0 0 0 0 7 0 9 5 0 8 4 0 0 8 7 0 0 4 2 9 0 3 3 4 0 7 0 0 2 5 0 4 1 1 1 0 3 1 6 0 9 5 0 4 1 1 0 0 5 5 6 0 2 5 0 0 0 8 7 0 8 8 0 0 4 0 1 9 3 0 8 8 0 9 6 8 0 0 7 0 3 1 9 0 7 9 0 5 8 0 8 8 7 0 2 0 0 0 9 9 0 0 0 9 0 2 0 0 2 7 2 0 1 6 0 0 2 2 9 0 0 0 8 0 5 2 2 0 9 1 7 0 5 0 0 0 7 6 1 0 4 6 6 0 4 3 3 1 0 1 2 3 0 2 0 0 3 3 2 0 7 2 4 0 8 5 0 9 6 8 0 0 0 0 5 0 5 3 0 0 0 3 0 0 4 3 0 2 8 3 0 9 9 0 3 8 0 2 5 8 0 3 8 0 6 9 0 2 6 0 0 1 3 0 4 4 2 0 9 2 7 6 0 0 0 2 0 0 2 0 4 6 0 8 5 0 0 6 5 2 0 9 1 0 8 0 0 7 2 5 0 8 6 0 5 2 8 0 2 6 3 0 4 9 0 3 2 7 0 6 4 5 8 0 0 9 0 1 7 6 1 0 8 0 0 0 3 3 0 0 8 0 7 0 0 0 0 6 6 6 2 0 0 3 8 0 7 0 0 1 7 0 0 7 5 0 4 1 4 0 6 3 2 0 2 7 0 5 2 0 2 2 0 0 0 6 6 0 8 7 0 8 4 3 0 0 9 6 0 0 0 3 0 0 9 0 6 0 0 0 3 4 4 0 1 1 1 1 0 8 9 0 2 5 0 8 9 3 8 0 1 3 3 0 1 0 0 4 1 3 0 4 5 0 0 2 1 0 0 3 0 0 5 0 6 0 0 7 0 0 6 5 0 7 7 0 0 3 8 4 0 3 5 0 1 2 5 3 0 3 6 7 3 0 2 7 2 0 9 6 1 0 2 9 0 0 2 0 0 0 9 0 8 2 0 0 8 7 5 0 4 5 3 0 4 7 7 0 0 5 1 2 0 9 4 0 2 8 0 9 1 4 0 3 9 0 0 0 3 2 0 7 6 0 5 8 1 0 5 2 0 0 0 0 3 0 2 3 8 0 0 4 0 1 4 0 0 4 3 0 7 9 7 0 0 5 0 7 9 5 9 0 3 8 3 0 6 5 1 0 0 5 1 0 1 6 0 0 5 5 0 9 9 5 8 0 1 5 5 0 0 0 8 3 0 0 1 3 0 8 3 0 6 4 0 0 5 0 6 2 9 0 1 3 0 0 4 0 8 4 0 0 0 9 7 0 1 3 0 0 0 6 5 0 5 2 0 1 3 7 0 3 7 0 9 6 7 0 9 9 2 0 5 1 4 0 6 4 7 5 0 0 5 4 0 3 0 0 8 4 7 0 5 0 0 5 8 0 9 4 0 8 1 0 0 2 0 2 4 7 0 3 0 0 0 3 4 3 3 0 6 9 0 0 9 0 6 9 3 0 7 0 0 0 0 3 6 5 0 0 3 5 7 0 4 3 9 0 9 0 0 0 7 2 7 0 1 4 0 0 1 0 0 0 4 2 0 0 7 0 0 6 4 0 0 5 3 0 3 7 3 0 9 1 0 1 4 0 1 0 0 0 0 4 7 4 5 0 8 0 0 0 6 0 4 5 0 0 2 5 0 0 7 5 1 6 0 7 6 2 0 9 7 0 1 2 0 5 8 1 0 0 0 5 0 0 0 3 0 3 3 0 3 8 3 0 5 9 9 0 6 9 0 9 5 0 7 9 2 4 0 5 4 3 0 0 3 9 0 0 8 5 0 2 2 0 0 5 0 5 6 0 0 9 7 0 4 4 0 0 3 0 3 4 0 4 9 0 0 0 3 0 6 0 0 8 7 0 0 5 1 0 3 4 5 0 2 4 0 0 0 0 4 3 0 6 9 9 0 1 5 6 0 1 1 7 0 8 4 2 4 0 6 9 1 6 0 4 9 9 2 0 4 7 0 7 5 0 8 0 0 0 5 0 0 5 6 4 0 9 2 0 6 6 7 0 0 3 3 0 8 5 0 0 8 0 8 7 0 8 0 0 4 8 0 0 0 2 0 0 0 2 9 3 0 0 4 0 6 9 0 0 5 1 0 0 6 0 0 2 0 9 1 1 0 8 1 9 2 0 0 0 0 7 0 7 7 4 0 0 0 5 0 1 6 0 0 5 0 7 1 4 0 7 8 0 8 0 0 6 4 4 5 0 1 9 0 0 2 0 4 1 0 6 6 0 5 1 9 0 2 2 4 0 6 9 0 9 2 0 7 8 5 0 8 6 0 0 0 5 9 0 0 0 0 1 0 4 8 0 0 8 6 7 9 0 9 4 0 4 4 8 0 0 7 8 5 0 0 4 0 0 8 9 0 5 3 0 4 2 0 9 5 5 3 0 8 2 0 4 5 0 0 4 5 0 6 4 0 4 2 4 0 9 8 4 4 0 1 6 0 0 0 3 0 6 5 1 0 7 3 0 0 7 5 0 3 5 9 0 0 8 1 0 4 7 0 1 9 7 0 1 4 1 0 2 5 0 7 5 0 9 6 9 0 0 6 3 9 0 0 7 7 0 1 9 1 0 1 3 0 0 7 3 7 0 6 2 9 3 0 0 0 2 1 0 7 2 9 0 5 3 5 0 7 4 4 0 6 6 0 5 1 7 0 2 0 0 0 9 1 8 0 7 8 0 4 2 8 0 2 8 0 6 4 0 7 1 0 0 0 1 0 2 1 2 0 0 6 7 0 0 1 2 0 8 1 8 0 0 0 3 4 0 4 5 0 2 1 9 0 3 4 7 0 9 9 6 0 2 0 0 3 7 2 6 0 5 0 0 0 0 0 6 0 0 3 5 0 8 7 3 0 0 3 0 3 4 8 0 1 3 0 0 4 4 1 0 8 3 8 8 0 9 5 0 6 2 7 0 8 6 0 2 2 0 0 0 0 9 0 4 2 9 0 1 1 3 0 1 1 0 3 5 0 0 0 3 0 0 0 4 0 7 2 9 0 2 6 0 5 6 4 0 9 1 0 0 5 3 0 6 7 2 9 0 0 3 1 0 0 7 6 0 4 9 0 7 5 8 1 0 3 5 5 0 0 4 0 0 7 0 9 1 0 0 0 0 9 4 0 6 0 0 0 5 3 4 0 6 8 0 9 7 3 7 0 0 7 6 0 0 0 4 0 9 3 0 5 8 5 0 2 7 5 0 1 1 0 1 5 3 0 5 4 0 0 0 0 9 0 5 1 0 0 4 5 2 0 0 0 7 0 9 2 0 0 8 0 9 2 0 0 2 1 0 7 0 0 0 4 0 7 1 5 0 2 1 1 0 0 0 4 0 3 9 0 0 3 4 0 0 7 5 1 1 0 7 1 6 0 5 9 0 0 0 4 5 0 7 5 0 4 7 0 7 6 0 9 3 0 8 3 1 7 0 5 5 0 9 0 0 7 9 0 1 6 0 6 7 6 0 4 7 7 6 0 0 8 0 4 8 0 8 3 4 7 0 7 1 6 0 0 6 7 8 0 8 2 0 0 1 0 0 0 0 3 3 0 0 4 6 0 6 1 3 0 7 8 0 0 3 4 9 0 8 6 9 5 0 3 8 0 0 0 0 9 0 9 5 0 0 2 3 0 9 9 3 8 0 0 0 2 0 0 6 0 1 8 0 0 4 0 0 5 9 0 4 7 0 5 5 0 8 3 0 0 4 8 0 0 7 0 0 0 8 0 1 6 0 1 8 0 7 4 0 6 0 0 8 0 0 4 5 0 6 2 3 0 2 8 0 4 2 0 9 9 0 6 8 8 7 0 1 3 8 0 0 2 0 9 3 5 0 8 4 0 0 7 7 0 8 7 9 0 0 2 0 2 4 2 8 0 6 0 0 0 8 2 2 0 5 0 0 8 5 2 1 0 9 3 1 0 0 2 0 0 3 7 8 0 1 5 0 0 4 4 3 0 7 6 8 0 3 6 0 8 2 9 0 1 0 0 2 8 4 3 0 0 2 0 4 7 6 0 4 8 0 3 9 0 8 7 0 2 6 0 1 2 4 0 0 0 0 7 0 4 7 7 0 7 3 5 0 1 8 0 9 2 0 8 0 0 0 2 0 0 0 8 9 0 4 1 0 2 7 6 0 1 6 6 0 6 5 4 0 0 6 3 0 0 0 9 0 8 9 0 0 6 0 9 3 0 4 9 0 2 8 8 2 0 5 3 0 7 7 3 2 0 7 6 0 0 9 0 2 7 5 0 0 9 5 0 1 2 0 4 2 9 2 0 9 4 6 0 0 1 0 1 4 0 7 3 2 0 6 5 0 7 5 0 9 9 5 0 6 6 0 2 7 0 0 0 0 8 3 5 0 5 4 0 5 8 0 9 2 0 0 4 1 0 5 3 0 6 6 0 7 2 5 3 0 7 5 0 8 0 0 4 4 0 7 6 2 0 0 5 0 3 5 9 0 0 9 0 0 0 7 3 6 8 0 0 9 0 4 2 0 3 7 0 6 7 9 1 0 3 7 4 0 8 6 0 1 0 0 0 4 5 0 5 5 4 0 5 7 4 0 9 7 0 0 4 4 0 5 3 2 0 6 0 0 1 4 0 1 4 0 6 2 0 0 3 4 0 0 2 0 0 0 0 6 0 1 2 0 5 0 0 0 7 0 2 9 2 0 2 9 0 3 5 4 3 0 3 9 0 8 8 0 2 3 4 0 0 2 4 0 9 1 0 4 4 0 7 7 1 0 6 8 0 7 7 0 2 3 0 0 2 6 7 0 8 0 0 0 0 6 2 0 0 4 6 0 2 8 0 0 9 6 1 0 5 8 0 8 3 0 4 7 0 9 1 8 6 0 9 5 1 0 6 5 0 0 0 0 5 9 0 9 1 0 0 0 4 4 0 7 8 6 1 0 9 4 1 0 4 0 0 0 3 2 0 7 0 0 8 2 0 4 7 6 3 0 6 7 0 6 4 0 0 0 0 8 4 0 9 4 0 2 2 0 2 6 0 7 4 0 0 8 1 0 0 5 4 3 0 0 3 0 4 6 0 8 5 1 0 0 0 8 0 0 4 2 0 0 9 0 5 3 0 0 3 8 0 0 3 4 0 7 4 4 0 3 1 0 1 3 0 8 5 1 2 0 1 4 0 7 6 6 0 2 2 0 7 8 8 0 1 6 0 0 0 5 1 0 5 3 0 0 0 0 8 2 0 0 6 1 0 0 6 1 0 1 3 3 0 2 5 0 3 2 9 9 0 5 4 5 0 7 7 0 8 7 7 0 7 9 0 1 3 2 5 0 9 3 0 4 7 2 0 0 2 0 6 0 0 0 2 0 9 3 1 0 0 5 2 9 0 8 2 9 0 5 9 0 6 2 8 1 0 9 4 0 0 0 9 0 5 0 0 7 8 4 0 6 7 0 0 5 0 4 9 0 2 1 0 7 4 8 7 0 5 8 0 0 4 5 0 8 4 7 0 8 3 5 0 4 7 0 0 9 9 8 0 6 4 5 0 1 0 0 8 5 0 0 0 5 4 0 6 4 0 0 0 9 6 0;
  |     1 0 0 0 0 0 0 0 0 0 0 0 1 0 0 0 0 0 0 0 0 0 0 1 0 0 0 0 0 0 0 0 0 0 0 0 1 0 0 0 0 0 0 0 0 0 0 0 0 0 0 0 0 0 1 0 0 0 0 0 0 0 0 0 0 0 0 0 0 0 0 0 0 0 0 0 0 0 0 1 0 0 1 0 0 1 0 0 0 0 0 1 0 0 0 0 0 0 0 0 0 0 1 0 0 0 0 0 0 1 0 0 0 0 0 0 1 0 0 0 0 0 0 0 0 0 0 0 0 1 0 0 0 1 0 0 0 0 0 1 0 0 0 1 0 0 0 0 0 0 0 0 0 0 0 0 0 0 0 0 0 0 0 1 0 0 0 0 0 1 0 0 0 1 0 0 0 0 0 0 1 0 0 1 0 0 1 0 0 0 0 0 0 0 0 0 0 0 0 1 0 0 0 0 0 0 0 1 0 0 1 0 0 0 0 0 0 0 0 0 0 0 0 0 0 0 0 0 1 0 0 0 0 0 0 0 0 0 0 1 0 0 1 0 0 0 1 0 0 0 0 0 0 0 0 0 0 0 1 0 0 0 0 0 0 1 0 0 0 0 0 1 0 0 0 1 0 0 0 0 0 0 0 0 0 0 1 0 0 0 0 0 0 0 1 0 0 0 0 0 0 0 1 0 0 0 1 0 0 0 1 0 0 1 0 0 1 0 0 1 0 0 1 0 0 0 0 0 0 0 0 0 0 0 0 0 0 0 0 0 0 0 0 0 1 0 0 0 0 0 0 0 0 0 0 0 0 0 0 0 0 0 0 0 0 1 0 0 0 0 0 0 0 0 0 0 0 1 0 0 0 1 0 0 0 1 0 0 0 1 0 0 0 1 0 0 0 1 0 0 0 0 0 0 0 1 0 0 0 1 0 0 0 0 0 1 0 0 1 0 0 0 1 0 0 1 0 0 0 0 0 0 0 1 0 0 0 1 0 0 0 1 0 0 1 0 0 0 0 0 0 1 0 0 1 0 0 0 0 0 0 0 1 0 0 0 1 0 0 0 0 0 0 1 0 0 1 0 0 0 1 0 0 1 0 0 0 0 0 0 0 0 0 0 0 0 0 1 0 0 0 0 0 0 0 0 0 0 0 0 1 0 0 1 0 0 0 0 0 0 0 1 0 0 0 0 0 0 1 0 0 0 0 0 0 0 0 0 0 0 0 1 0 0 0 0 0 0 0 0 0 0 0 0 0 1 0 0 0 0 0 0 0 0 0 0 0 0 0 0 0 1 0 0 1 0 0 0 0 0 0 0 0 0 0 0 0 0 0 0 0 1 0 0 1 0 0 0 0 0 0 1 0 0 0 0 0 0 0 0 0 0 0 0 0 0 0 0 0 0 0 0 0 0 0 0 0 0 0 0 1 0 0 0 1 0 0 0 0 0 0 0 0 0 1 0 0 1 0 0 0 0 0 0 0 1 0 0 1 0 0 0 1 0 0 1 0 0 1 0 0 0 0 0 0 0 1 0 0 0 1 0 0 1 0 0 0 0 0 0 0 0 0 1 0 0 0 1 0 0 0 0 0 0 0 0 0 0 0 0 0 0 0 0 1 0 0 0 0 0 0 0 0 0 0 0 0 0 1 0 0 0 1 0 0 1 0 0 0 0 0 0 0 0 0 0 0 1 0 0 0 0 0 0 0 1 0 0 1 0 0 0 0 0 1 0 0 1 0 0 0 0 0 0 0 0 0 0 0 0 0 0 0 0 1 0 0 0 1 0 0 0 1 0 0 0 0 0 0 0 1 0 0 0 0 0 0 1 0 0 1 0 0 0 0 0 0 0 0 1 0 0 0 0 0 0 1 0 0 0 0 0 0 0 1 0 0 0 1 0 0 0 1 0 0 1 0 0 0 0 0 0 0 0 0 0 0 1 0 0 0 0 0 0 0 0 1 0 0 0 0 0 0 0 0 0 0 0 0 1 0 0 0 1 0 0 0 0 0 0 0 0 0 0 0 0 0 0 0 1 0 0 1 0 0 1 0 0 0 1 0 0 0 0 0 1 0 0 0 0 0 0 0 1 0 0 0 0 0 0 0 0 0 0 0 0 1 0 0 0 0 0 0 0 0 0 0 0 0 1 0 0 0 0 0 0 0 0 0 0 0 0 0 0 0 0 0 0 0 0 1 0 0 0 0 0 1 0 0 1 0 0 1 0 0 0 1 0 0 0 0 0 0 0 0 1 0 0 0 0 0 0 0 0 1 0 0 0 0 0 0 1 0 0 0 0 0 0 0 0 0 0 0 1 0 0 0 0 0 0 0 0 0 0 0 0 0 0 0 1 0 0 0 0 0 0 0 0 0 0 0 0 0 0 1 0 0 0 0 0 0 1 0 0 1 0 0 1 0 0 0 0 0 0 0 1 0 0 0 0 0 0 1 0 0 1 0 0 0 1 0 0 0 1 0 0 1 0 0 0 1 0 0 0 0 0 0 0 0 0 0 0 0 0 0 0 1 0 0 0 0 0 0 1 0 0 0 0 0 0 0 0 0 0 0 0 0 0 1 0 0 0 0 0 0 0 0 0 0 0 0 0 1 0 0 0 1 0 0 1 0 0 0 0 0 0 0 0 0 0 1 0 0 0 0 0 0 0 0 0 0 0 0 0 0 0 0 0 1 0 0 0 0 0 1 0 0 1 0 0 0 0 0 0 0 0 0 0 0 0 0 0 0 0 0 0 0 0 0 0 0 0 0 0 1 0 0 0 1 0 0 1 0 0 0 0 0 0 0 1 0 0 1 0 0 1 0 0 0 0 0 0 0 0 1 0 0 0 1 0 0 0 0 0 0 0 0 0 0 1 0 0 0 0 0 0 0 0 0 0 0 1 0 0 0 1 0 0 0 1 0 0 0 0 0 0 1 0 0 0 0 0 0 0 0 0 1 0 0 0 1 0 0 1 0 0 0 1 0 0 1 0 0 0 0 0 0 1 0 0 0 1 0 0 0 0 0 0 1 0 0 1 0 0 0 1 0 0 0 1 0 0 0 0 0 0 0 1 0 0 0 1 0 0 0 0 0 0 0 0 0 0 0 0 0 0 0 0 0 0 0 0 1 0 0 0 0 0 0 1 0 0 0 1 0 0 0 1 0 0 0 0 0 0 0 1 0 0 0 0 0 0 0 0 0 0 0 1 0 0 0 0 0 0 1 0 0 1 0 0 0 0 0 0 1 0 0 1 0 0 0 0 0 0 1 0 0 1 0 0 0 0 0 0 0 0 0 0 0 0 1 0 0 0 0 0 1 0 0 0 0 0 0 0 0 0 0 0 0 0 1 0 0 0 0 0 0 0 0 0 0 0 0 0 0 0 0 0 1 0 0 0 0 0 0 0 0 0 0 0 0 0 0 0 0 0 0 0 0 1 0 0 1 0 0 0 0 0 0 0 0 0 0 0 0 1 0 0 0 1 0 0 1 0 0 1 0 0 0 1 0 0 0 0 0 0 0 1 0 0 1 0 0 1 0 0 0 0 0 0 0 0 0 0 1 0 0 0 1 0 0 0 1 0 0 0 0 0 0 1 0 0 0 1 0 0 0 0 0 0 0 0 0 0 0 0 0 0 0 0 0 0 0 1 0 0 0 1 0 0 1 0 0 0 0 0 0 0 0 0 0 1 0 0 1 0 0 1 0 0 0 0 0 0 0 0 1 0 0 0 1 0 0 0 1 0 0 0 0 0 0 0 0 0 0 0 0 1 0 0 0 0 0 0 0 1 0 0 0 1 0 0 1 0 0 0 0 0 0 0 0 0 0 1 0 0 0 0 0 0 0 0 1 0 0 0 1 0 0 1 0 0 1 0 0 0 0 0 0 0 0 0 0 0 1 0 0 1 0 0 0 1 0 0 0 0 0 0 0 1 0 0 0 1 0 0 0 0 0 0 0 0 0 1 0 0 0 1 0 0 0 0 0 0 0 0 0 0 0 0 0 0 0 1 0 0 0 1 0 0 1 0 0 0 0 0 0 0 0 1 0 0 0 0 0 0 0 0 1 0 0 0 1 0 0 0 0 0 1 0 0 0 0 0 0 1 0 0 1 0 0 1 0 0 0 0 0 0 0 0 0 0 0 0 0 0 0 1 0 0 0 0 0 0 1 0 0 1 0 0 0 0 0 0 0 1 0 0 0 0 0 0 0 0 1 0 0 0 1 0 0 0 0 0 0 0 0 0 0 0 0 0 0 0 1 0 0 1 0 0 0 0 0 0 1 0 0 0 0 0 0 0 0 1 0 0 0 0 0 1 0 0 0 0 0 0 0 0 0 0 0 0 0 0 0 0 0 0 0 0 0 0 0 0 0 0 0 0 0 0 0 0 0 1 0 0 0 1 0 0 0 1 0 0 0 0 0 0 1 0 0 0 0 0 0 1 0 0 0 0 0 0 0 0 0 0 0 0 0 0 0 1 0 0 1 0 0 1 0 0 0 0 0 0 0 0 0 0 0 0 1 0 0 0 0 0 0 1 0 0 1 0 0 0 0 0 0 0 1 0 0 0 0 0 0 0 0 0 0 0 0 0 0 1 0 0 1 0 0 0 0 0 0 0 1 0 0 0 1 0 0 0 0 0 0 0 0 0 0 1 0 0 0 0 0 0 0 0 0 1 0 0 1 0 0 0 0 0 0 0 0 0 0 0 0 1 0 0 1 0 0 0 1 0 0 0 0 0 0 0 0 0 0 0 1 0 0 0 1 0 0 0 1 0 0 0 0 0 0 0 0 0 0 0 0 0 0 0 0 0 0 0 0 0 0 0 0 0 0 0 0 1 0 0 0 1 0 0 1 0 0 0 1 0 0 1 0 0 0 1 0 0 0 0 0 0 1 0 0 1 0 0 1 0 0 0 0 0 0 0 1 0 0 0 0 0 0 0 0 0 0 0 0 0 0 1 0 0 0 0 0 1 0 0 1 0 0 0 0 0 0 0 0 0 0 0 0 0 1 0 0 0 1 0 0 0 1 0 0 1 0 0 1 0 0 0 0 0 0 0 0 0 0 0 0 0 0 0 0 0 1 0 0 1 0 0 0 0 0 1 0 0 0 1 0 0 0 1 0 0 1 0 0 1 0 0 0 1 0 0 0 0 0 0 0 0 0 0 0 0 1 0 0 0 0 0 0 0 0 1 0 0 0 0 0 0 0 0 0 0 0 1 0 0 1 0 0 0 1 0 0 1 0 0 0 0 0 0 0 1 0 0 1 0 0 1 0 0 0 1 0 0 1 0 0 0 0 0 0 0 0 1 0 0 0 0 0 0 1 0 0 0 1 0 0 0 0 0 0 0 0 0 0 0 0 0 0 1 0 0 1 0 0 0 0 0 0 0 1 0 0 1 0 0 0 0 0 0 0 0 0 0 0 0 0 0 0 1 0 0 0 0 0 0 0 0 0 0 0 0 0 0 0 0 0 0 0 0 0 0 0 0 0 1 0 0 0 0 0 0 0 0 0 0 1 0 0 0 1 0 0 0 1 0 0 0 0 0 0 1 0 0 0 1 0 0 0 0 0 0 0 0 0 0 0 0 1 0 0 0 0 0 0 0 1 0 0 0 1 0 0 0 0 0 0 0 0 1 0 0 0 0 0 0 1 0 0 0 1 0 0 0 0 0 0 0 0 0 0 0 1 0 0 0 1 0 0 0 1 0 0 0 1 0 0 0 0 0 0 1 0 0 0 1 0 0 0 1 0 0 0 0 0 0 0 0 0 0 0 1 0 0 0 1 0 0 1 0 0 0 1 0 0 0 1 0 0 0 0 0 0 0 1 0 0 1 0 0 0 1 0 0 1 0 0 0 1 0 0 0 0 0 0 0 0 0 0 0 0 0 0 0 0 0 0 0 0 0 0 1 0 0 0 0 0 0 0 1 0 0 0 0 0 0 0 0 0 0 0 0 0 0 1 0 0 0 0 0 0 0 1 0 0 0 1 0 0 0 1 0 0 0 1 0 0 0 0 0 0 0 0 0 0 0 0 0 0 0 1 0 0 1 0 0 0 0 0 0 0 0 0 0 1 0 0 0 0 0 0 0 0 0 0 0 1 0 0 0 0 0 0 0 0 0 0 0 0 0 0 0 0 0 0 0 0 0 0 0 0 0 0 0 0 0 0 1 0 0 0 1 0 0 0 1 0 0 0 1 0 0 0 1 0 0 0 0 0 0 0 0 0 0 0 0 0 0 0 0 0 0 0 0 1 0 0 0 0 0 0 0 0 1 0 0 0 0 0 0 0 1 0 0 1 0 0 1 0 0 1 0 0 0 0 0 0 0 0 0 0 0 1 0 0 0 0 0 0 0 0 0 0 0 0 0 0 0 0 0 0 0 1 0 0 0 0 0 0 0 0 1 0 0 1 0 0 0 1 0 0 0 1 0 0 0 0 0 0 0 0 0 0 0 0 0 0 0 0 1 0 0 0 1 0 0 0 1 0 0 0 0 0 0 0 1 0 0 0 0 0 0 1 0 0 0 0 0 0 0 0 0 1 0 0 1 0 0 1 0 0 0 0 0 0 0 0 0 0 0 0 0 1 0 0 0 0 0 1 0 0 0 0 0 1 0 0 1 0 0 0 0 0 0 1 0 0 0 0 0 1 0 0 0 0 0 0 0 1 0 0 0 1 0 0 1 0 0 0 0 0 0 0 0 0 0 1 0 0 0 1 0 0 0 0 0 0 0 1 0 0 0 0 0 0 0 1 0 0 0 0 0 0 0 1 0 0 0 1 0 0 0 0 0 0 0 1 0 0 0 1 0 0 0 0 0 0 0 0 0 0 0 0 0 0 0 0 0 0 0 0 0 0 0 0 0 1 0 0 0 1 0 0 1 0 0 1 0 0 0 0 0 1 0 0 0 0 0 0 0 0 0 0 0 0 1 0 0 0 1 0 0 1 0 0 1 0 0 0 1 0 0 0 1 0 0 1 0 0 1 0 0 0 0 0 0 0 1 0 0 0 0 0 0 0 1 0 0 0 0 0 0 1 0 0 1 0 0 1 0 0 0 0 0 0 0 0 0 0 0 0 0 0 0 1 0 0 0 0 0 0 0 0 0 0 1 0 0 1 0 0 0 0 0 0 0 0 0 0 0 0 0 0 0 0 0 1 0 0 0 1 0 0 0 0 0 1 0 0 0 1 0 0 0 0 0 0 0 0 0 0 0 0 1 0 0 1 0 0 1 0 0 0 1 0 0 1 0 0 1 0 0 0 0 0 0 0 0 0 0 0 0 0 1 0 0 1 0 0 0 1 0 0 0 0 0 0 0 1 0 0 0 0 0 0 0 0 0 0 0 1 0 0 0 0 0 0 0 0 0 0 1 0 0 0 0 0 0 1 0 0 1 0 0 0 1 0 0 0 0 0 0 0 1 0 0 1 0 0 0 1 0 0 0 1 0 0 1 0 0 0 0 0 1 0 0 0 0 0 0 1 0 0 0 0 0 0 0 1 0 0 0 0 0 1 0 0 1 0 0 0 1 0 0 0 0 0 0 0 1 0 0 0 0 0 1 0 0 0 1 0 0 0 0 0 0 0 0 0 1 0 0 0 1 0 0 0 0 0 1 0 0 0 1 0 0 0 0 0 0 0 0 1 0 0 1 0 0 0 1 0 0 0 0 0 0 0 1 0 0 0 0 0 0 0 0 0 0 0 0 0 1 0 0 0 0 0 0 0 0 0 0 0 0 1 0 0 0 0 0 0 0 0 0 0 0 0 1 0 0 0 1 0 0 0 0 0 0 1 0 0 0 0 0 0 0 0 0 0 1 0 0 1 0 0 0 0 0 0 0 0 1 0 0 1 0 0 1 0 0 1 0 0 0 0 0 0 0 1 0 0 0 0 0 0 1 0 0 1 0 0 0 0 0 0 0 1 0 0 0 0 0 0 1 0 0 0 0 0 0 0 0 0 0 1 0 0 0 0 0 0 1 0 0 0 0 0 0 0 1 0 0 1 0 0 0 1 0 0 0 0 0 0 1 0 0 0 0 0 0 0 0 0 0 0 0 1 0 0 0 1 0 0 0 1 0 0 0 1 0 0 0 1 0 0 0 0 0 0 0 1 0 0 0 0 0 0 0 0 0 0 1 0 0 0 0 0 0 0 1 0 0 1 0 0 0 1 0 0 0 0 0 1 0 0 0 0 0 0 0 0 0 0 0 0 0 0 0 0 0 0 0 0 0 0 0 0 0 0 1 0 0 0 0 0 0 1 0 0 0 0 0 0 1 0 0 0 0 0 1 0 0 0 0 0 0 0 0 0 0 0 0 0 0 1 0 0 0 1 0 0 0 1 0 0 0 0 0 0 0 1 0 0 0 1 0 0 0 0 0 0 0 0 0 0 1 0 0 0 0 0 0 0];
undefined symbols (not defined in the file): DiscIntNeverNeededParam
libraries: simulink x2
settings Model: Creator=pete  LastModifiedBy=pete

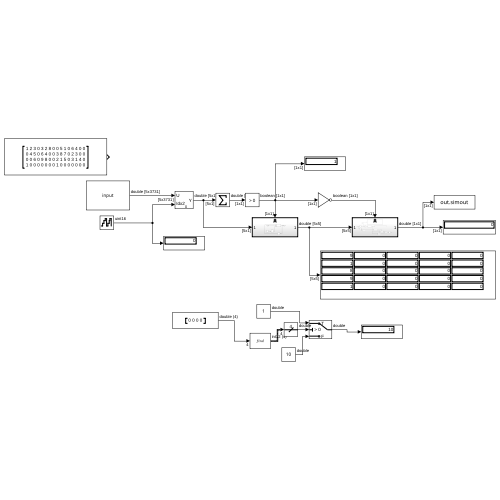
[thumbnail: Simulink's stored preview of the top-level diagram]
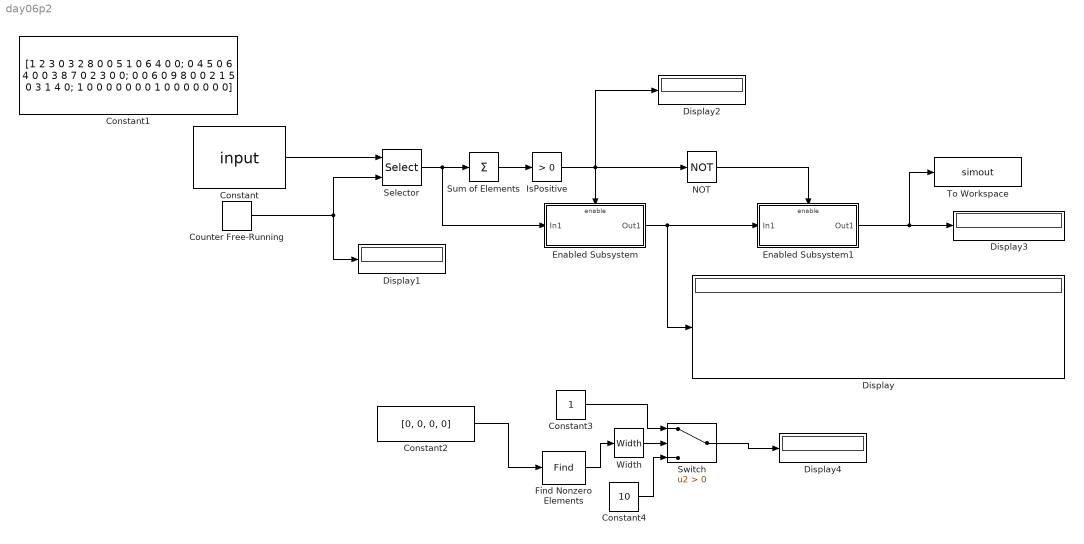
== system day06p2 ==
  Constant : Constant  Value=input
  Constant1 : Constant  Value=|
      | [1 2 3 0 3 2 8 0 0 5 1 0 6 4 0 0;
      | 0 4 5 0 6 4 0 0 3 8 7 0 2 3 0 0;
      | 0 0 6 0 9 8 0 0 2 1 5 0 3 1 4 0;
      | 1 0 0 0 0 0 0 0 1 0 0 0 0 0 0 0]
  Constant2 : Constant  Value=[0, 0, 0, 0]
  Constant3 : Constant
  Constant4 : Constant  Value=10
  Counter Free-Running : simulink/Sources/Counter Free-Running  NumBits=16  tsamp=-1
  Display{,1..4} (5 alike) : Display
  Enabled Subsystem : Subsystem  TreatAsAtomicUnit=on
  Enabled Subsystem1 : Subsystem  TreatAsAtomicUnit=on
  Find Nonzero Elements : Find  NumberOfInputDimensions=3  IndexMode=Zero-based
  IsPositive : simulink/Logic and Bit Operations/Compare To Zero  relop=>  OutDataTypeStr=boolean
      settings: LibrarySourceBlock=|
      | simulink/Quick Insert/Logic and Bit
      | Operations/IsPositive
  NOT : Logic  Operator=NOT  IconShape=distinctive  AllPortsSameDT=off  OutDataTypeStr=boolean
  Selector : Selector  NumberOfDimensions=2  IndexMode=Zero-based  InputPortWidth=3  IndexOptions=Index vector (dialog),Index vector (port)  Indices=[0:4],1  OutputSizes=1,1
  Sum of Elements : Sum  Inputs=+
  Switch : Switch  Criteria=u2 > Threshold  SaturateOnIntegerOverflow=off  InputSameDT=off
  To Workspace : ToWorkspace  VariableName=simout  SaveFormat=Timeseries  SampleTime=-1
  Width : Width
  wires:
  Constant/1 -> Selector/1
  Counter Free-Running/1 -> Display1/1, Selector/2
  Selector/1 -> Enabled Subsystem/1(In1), Sum of Elements/1
  Sum of Elements/1 -> IsPositive/1
  IsPositive/1 -> NOT/1, Enabled Subsystem/Enable, Display2/1
  Enabled Subsystem/1(Out1) -> Enabled Subsystem1/1(In1), Display/1
  NOT/1 -> Enabled Subsystem1/Enable
  Enabled Subsystem1/1(Out1) -> To Workspace/1, Display3/1
  Constant2/1 -> Find Nonzero Elements/1
  Find Nonzero Elements/1 -> Width/1
  Constant3/1 -> Switch/1
  Constant4/1 -> Switch/3
  Switch/1 -> Display4/1
  Width/1 -> Switch/2

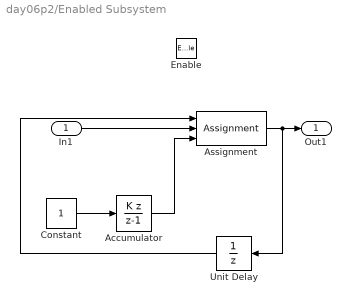
== system day06p2/Enabled Subsystem ==
  In1 : Inport
  Enable : EnablePort  StatesWhenEnabling=reset
  Accumulator : DiscreteIntegrator  IntegratorMethod=Accumulation: Backward Euler  SampleTime=-1  ICPrevOutput=DiscIntNeverNeededParam  ICPrevScaledInput=DiscIntNeverNeededParam
  Assignment : Assignment  NumberOfDimensions=2  DiagnosticForDimensions=Warning  IndexOptions=Index vector (dialog),Index vector (port)  Indices=[1:5],1  OutputSizes=1,1
  Constant : Constant
  Unit Delay : UnitDelay  SampleTime=-1
  Out1 : Outport  InitialOutput=zeros(5, 5)
  wires:
  Constant/1 -> Accumulator/1
  Assignment/1 -> Unit Delay/1, Out1/1
  Accumulator/1 -> Assignment/3
  In1/1 -> Assignment/2
  Unit Delay/1 -> Assignment/1

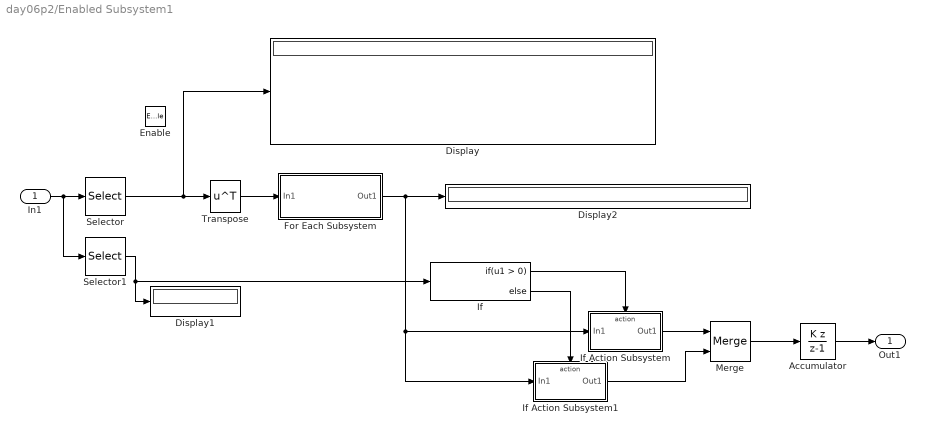
== system day06p2/Enabled Subsystem1 ==
  In1 : Inport
  Enable : EnablePort  PropagateVarSize=During execution
  Accumulator : DiscreteIntegrator  IntegratorMethod=Accumulation: Backward Euler  SampleTime=-1  ICPrevOutput=DiscIntNeverNeededParam  ICPrevScaledInput=DiscIntNeverNeededParam
  Display : Display
  Display1 : Display
  Display2 : Display
  For Each Subsystem : Subsystem  TreatAsAtomicUnit=on
  If : If
  If Action Subsystem : Subsystem  TreatAsAtomicUnit=on
  If Action Subsystem1 : Subsystem  TreatAsAtomicUnit=on
  Merge : Merge
  Selector : Selector  NumberOfDimensions=2  InputPortWidth=3  IndexOptions=Index vector (dialog),Index vector (dialog)  Indices=[1:4],[1:4]  OutputSizes=1,1
  Selector1 : Selector  NumberOfDimensions=2  InputPortWidth=3  IndexOptions=Index vector (dialog),Index vector (dialog)  Indices=5,1  OutputSizes=1,1
  Transpose : Math  Operator=transpose
  Out1 : Outport
  wires:
  In1/1 -> Selector1/1, Selector/1
  Selector/1 -> Transpose/1, Display/1
  Transpose/1 -> For Each Subsystem/1(In1)
  Selector1/1 -> If/1, Display1/1
  For Each Subsystem/1(Out1) -> If Action Subsystem1/1(In1), If Action Subsystem/1(In1), Display2/1
  If/1 -> If Action Subsystem/Action
  If/2 -> If Action Subsystem1/Action
  If Action Subsystem1/1(Out1) -> Merge/2
  Merge/1 -> Accumulator/1
  Accumulator/1 -> Out1/1
  If Action Subsystem/1(Out1) -> Merge/1

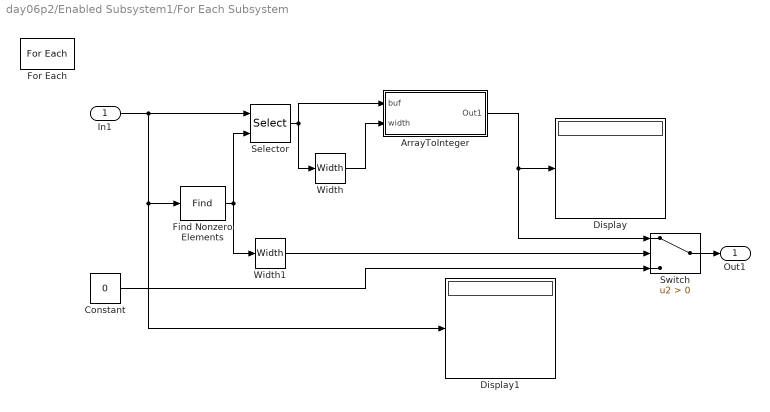
== system day06p2/Enabled Subsystem1/For Each Subsystem ==
  In1 : Inport  Partition=on  PartitionDimension=1  PartitionWidth=1  PartitionOffset=0
  ArrayToInteger : Subsystem  TreatAsAtomicUnit=on
  Constant : Constant  Value=0
  Display : Display
  Display1 : Display
  Find Nonzero Elements : Find  NumberOfInputDimensions=3  IndexMode=Zero-based
  For Each : ForEach  DisableCoverage=on
  Selector : Selector  IndexMode=Zero-based  InputPortWidth=4  IndexOptions=Index vector (port)  Indices=[1 3]  OutputSizes=1
  Switch : Switch  Criteria=u2 > Threshold  SaturateOnIntegerOverflow=off  InputSameDT=off
  Width : Width
  Width1 : Width
  Out1 : Outport  ConcatenationDimension=1
  wires:
  In1/1 -> Display1/1, Find Nonzero Elements/1, Selector/1
  Find Nonzero Elements/1 -> Selector/2, Width1/1
  Selector/1 -> ArrayToInteger/1(buf), Width/1
  Width/1 -> ArrayToInteger/2(width)
  ArrayToInteger/1(Out1) -> Switch/1, Display/1
  Width1/1 -> Switch/2
  Constant/1 -> Switch/3
  Switch/1 -> Out1/1

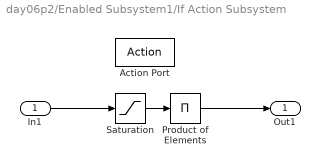
== system day06p2/Enabled Subsystem1/If Action Subsystem ==
  In1 : Inport
  Action Port : ActionPort  ActionPortLabel=if(u1 > 0)
  Product of Elements : Product  Inputs=*
  Saturation : Saturate  UpperLimit=Inf  LowerLimit=1
  Out1 : Outport
  wires:
  In1/1 -> Saturation/1
  Saturation/1 -> Product of Elements/1
  Product of Elements/1 -> Out1/1

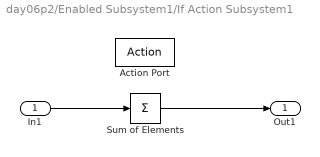
== system day06p2/Enabled Subsystem1/If Action Subsystem1 ==
  In1 : Inport
  Action Port : ActionPort  ActionPortLabel=else
  Sum of Elements : Sum  Inputs=+
  Out1 : Outport
  wires:
  In1/1 -> Sum of Elements/1
  Sum of Elements/1 -> Out1/1

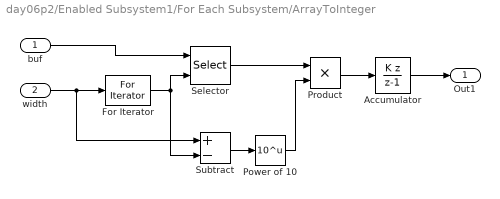
== system day06p2/Enabled Subsystem1/For Each Subsystem/ArrayToInteger ==
  buf : Inport
  width : Inport  Port=2
  Accumulator : DiscreteIntegrator  IntegratorMethod=Accumulation: Backward Euler  SampleTime=-1  ICPrevOutput=DiscIntNeverNeededParam  ICPrevScaledInput=DiscIntNeverNeededParam
  For Iterator : ForIterator  ResetStates=reset  IterationSource=external  IterationLimit=4
  Power of 10 : Math  Operator=10^u
  Product : Product
  Selector : Selector  InputPortWidth=4  IndexOptions=Index vector (port)  Indices=[1 3]  OutputSizes=1
  Subtract : Sum  Inputs=+-
  Out1 : Outport
  wires:
  width/1 -> Subtract/1, For Iterator/1
  buf/1 -> Selector/1
  For Iterator/1 -> Subtract/2, Selector/2
  Selector/1 -> Product/1
  Subtract/1 -> Power of 10/1
  Power of 10/1 -> Product/2
  Product/1 -> Accumulator/1
  Accumulator/1 -> Out1/1
